simulink model "SimulinkAnalysisofCheetahTail"  (R2022a)
(part 4 of 21)

t1922 = ct{753};
t1923 = ct{754};
t1924 = ct{755};
t1926 = ct{756};
t1928 = ct{757};
t1929 = ct{758};
t1930 = ct{759};
t1931 = ct{760};
t1933 = ct{761};
t1935 = ct{762};
t1937 = ct{763};
t1938 = ct{764};
t1939 = ct{765};
t1940 = ct{766};
t1941 = ct{767};
t1942 = ct{768};
t1943 = ct{769};
t1945 = ct{770};
t1949 = ct{771};
t195 = ct{772};
t1950 = ct{773};
t1951 = ct{774};
t1952 = ct{775};
t1953 = ct{776};
t1955 = ct{777};
t1956 = ct{778};
t1957 = ct{779};
t1959 = ct{780};
t1960 = ct{781};
t1961 = ct{782};
t1962 = ct{783};
t1963 = ct{784};
t1964 = ct{785};
t1965 = ct{786};
t1966 = ct{787};
t1967 = ct{788};
t1968 = ct{789};
t1969 = ct{790};
t197 = ct{791};
t1970 = ct{792};
t1971 = ct{793};
t1973 = ct{794};
t1974 = ct{795};
t1975 = ct{796};
t1976 = ct{797};
t1977 = ct{798};
t1978 = ct{799};
t1979 = ct{800};
t1980 = ct{801};
t1981 = ct{802};
t1982 = ct{803};
t1983 = ct{804};
t1984 = ct{805};
t1985 = ct{806};
t1986 = ct{807};
t1987 = ct{808};
t1988 = ct{809};
t1989 = ct{810};
t1990 = ct{811};
t1992 = ct{812};
t1993 = ct{813};
t1994 = ct{814};
t1995 = ct{815};
t1996 = ct{816};
t1998 = ct{817};
t1999 = ct{818};
t2 = ct{819};
t2000 = ct{820};
t2004 = ct{821};
t2005 = ct{822};
t2006 = ct{823};
t2007 = ct{824};
t2008 = ct{825};
t2009 = ct{826};
t2014 = ct{827};
t2015 = ct{828};
t2016 = ct{829};
t2017 = ct{830};
t2018 = ct{831};
t2020 = ct{832};
t2022 = ct{833};
t2023 = ct{834};
t2024 = ct{835};
t2025 = ct{836};
t2026 = ct{837};
t2027 = ct{838};
t2028 = ct{839};
t2030 = ct{840};
t2033 = ct{841};
t2035 = ct{842};
t2036 = ct{843};
t2037 = ct{844};
t2041 = ct{845};
t2042 = ct{846};
t2043 = ct{847};
t2045 = ct{848};
t2046 = ct{849};
t2047 = ct{850};
t2048 = ct{851};
t2049 = ct{852};
t2050 = ct{853};
t2052 = ct{854};
t2053 = ct{855};
t2056 = ct{856};
t2057 = ct{857};
t2058 = ct{858};
t2059 = ct{859};
t2060 = ct{860};
t2061 = ct{861};
t2062 = ct{862};
t2063 = ct{863};
t2064 = ct{864};
t2065 = ct{865};
t2066 = ct{866};
t2067 = ct{867};
t2068 = ct{868};
t2069 = ct{869};
t2070 = ct{870};
t2072 = ct{871};
t2074 = ct{872};
t2075 = ct{873};
t2076 = ct{874};
t2077 = ct{875};
t2078 = ct{876};
t2079 = ct{877};
t2081 = ct{878};
t2082 = ct{879};
t2083 = ct{880};
t2084 = ct{881};
t2087 = ct{882};
t2088 = ct{883};
t2090 = ct{884};
t2091 = ct{885};
t2092 = ct{886};
t2094 = ct{887};
t2095 = ct{888};
t2096 = ct{889};
t2097 = ct{890};
t2098 = ct{891};
t2099 = ct{892};
t2100 = ct{893};
t2102 = ct{894};
t2103 = ct{895};
t2104 = ct{896};
t2105 = ct{897};
t2106 = ct{898};
t2108 = ct{899};
t2109 = ct{900};
t2110 = ct{901};
t2113 = ct{902};
t2114 = ct{903};
t2116 = ct{904};
t2117 = ct{905};
t2118 = ct{906};
t2119 = ct{907};
t2120 = ct{908};
t2121 = ct{909};
t2123 = ct{910};
t2124 = ct{911};
t2126 = ct{912};
t2127 = ct{913};
t2129 = ct{914};
t2130 = ct{915};
t2131 = ct{916};
t2132 = ct{917};
t2134 = ct{918};
t2135 = ct{919};
t2136 = ct{920};
t2137 = ct{921};
t214 = ct{922};
t2141 = ct{923};
t2142 = ct{924};
t2143 = ct{925};
t2144 = ct{926};
t2146 = ct{927};
t2147 = ct{928};
t2148 = ct{929};
t2149 = ct{930};
t2150 = ct{931};
t2151 = ct{932};
t2152 = ct{933};
t2153 = ct{934};
t2154 = ct{935};
t2155 = ct{936};
t2156 = ct{937};
t2157 = ct{938};
t2158 = ct{939};
t2161 = ct{940};
t2163 = ct{941};
t2165 = ct{942};
t2167 = ct{943};
t2168 = ct{944};
t2171 = ct{945};
t2172 = ct{946};
t2174 = ct{947};
t2176 = ct{948};
t2178 = ct{949};
t2179 = ct{950};
t2181 = ct{951};
t2182 = ct{952};
t2183 = ct{953};
t2184 = ct{954};
t2186 = ct{955};
t2187 = ct{956};
t2188 = ct{957};
t2189 = ct{958};
t2190 = ct{959};
t2191 = ct{960};
t2192 = ct{961};
t2196 = ct{962};
t2199 = ct{963};
t2201 = ct{964};
t2202 = ct{965};
t2203 = ct{966};
t2205 = ct{967};
t2206 = ct{968};
t2208 = ct{969};
t2209 = ct{970};
t2211 = ct{971};
t2212 = ct{972};
t2213 = ct{973};
t2214 = ct{974};
t2215 = ct{975};
t2216 = ct{976};
t2217 = ct{977};
t2218 = ct{978};
t2219 = ct{979};
t2220 = ct{980};
t2221 = ct{981};
t2222 = ct{982};
t2223 = ct{983};
t2224 = ct{984};
t2225 = ct{985};
t2227 = ct{986};
t2228 = ct{987};
t2229 = ct{988};
t2230 = ct{989};
t2231 = ct{990};
t2232 = ct{991};
t2233 = ct{992};
t2235 = ct{993};
t2237 = ct{994};
t2238 = ct{995};
t2239 = ct{996};
t2240 = ct{997};
t2242 = ct{998};
t2245 = ct{999};
t2246 = ct{1000};
t2247 = ct{1001};
t2248 = ct{1002};
t2249 = ct{1003};
t2251 = ct{1004};
t2252 = ct{1005};
t2253 = ct{1006};
t2254 = ct{1007};
t2255 = ct{1008};
t2257 = ct{1009};
t2258 = ct{1010};
t2259 = ct{1011};
t2260 = ct{1012};
t2262 = ct{1013};
t2263 = ct{1014};
t2265 = ct{1015};
t2267 = ct{1016};
t2268 = ct{1017};
t2269 = ct{1018};
t2271 = ct{1019};
t2272 = ct{1020};
t2273 = ct{1021};
t2274 = ct{1022};
t2276 = ct{1023};
t2277 = ct{1024};
t2281 = ct{1025};
t2285 = ct{1026};
t2286 = ct{1027};
t2287 = ct{1028};
t2288 = ct{1029};
t2289 = ct{1030};
t2290 = ct{1031};
t2292 = ct{1032};
t2293 = ct{1033};
t2294 = ct{1034};
t2296 = ct{1035};
t2298 = ct{1036};
t2299 = ct{1037};
t2301 = ct{1038};
t2303 = ct{1039};
t2304 = ct{1040};
t2305 = ct{1041};
t2307 = ct{1042};
t2308 = ct{1043};
t2309 = ct{1044};
t2312 = ct{1045};
t2314 = ct{1046};
t2316 = ct{1047};
t2317 = ct{1048};
t2318 = ct{1049};
t2319 = ct{1050};
t2320 = ct{1051};
t2321 = ct{1052};
t2322 = ct{1053};
t2323 = ct{1054};
t2324 = ct{1055};
t2325 = ct{1056};
t2326 = ct{1057};
t2327 = ct{1058};
t2328 = ct{1059};
t2330 = ct{1060};
t2331 = ct{1061};
t2334 = ct{1062};
t2335 = ct{1063};
t2336 = ct{1064};
t2338 = ct{1065};
t2339 = ct{1066};
t2340 = ct{1067};
t2341 = ct{1068};
t2342 = ct{1069};
t2343 = ct{1070};
t2344 = ct{1071};
t2345 = ct{1072};
t2346 = ct{1073};
t2347 = ct{1074};
t2348 = ct{1075};
t2349 = ct{1076};
t2350 = ct{1077};
t2351 = ct{1078};
t2352 = ct{1079};
t2353 = ct{1080};
t2354 = ct{1081};
t2356 = ct{1082};
t2357 = ct{1083};
t2358 = ct{1084};
t2360 = ct{1085};
t2361 = ct{1086};
t2362 = ct{1087};
t2363 = ct{1088};
t2364 = ct{1089};
t2365 = ct{1090};
t2369 = ct{1091};
t2371 = ct{1092};
t2373 = ct{1093};
t2375 = ct{1094};
t2376 = ct{1095};
t2377 = ct{1096};
t2378 = ct{1097};
t2380 = ct{1098};
t2381 = ct{1099};
t2382 = ct{1100};
t2385 = ct{1101};
t2386 = ct{1102};
t2387 = ct{1103};
t2388 = ct{1104};
t2389 = ct{1105};
t2390 = ct{1106};
t2392 = ct{1107};
t2396 = ct{1108};
t2397 = ct{1109};
t2399 = ct{1110};
t24 = ct{1111};
t2400 = ct{1112};
t2401 = ct{1113};
t2403 = ct{1114};
t2404 = ct{1115};
t2406 = ct{1116};
t2407 = ct{1117};
t2408 = ct{1118};
t2409 = ct{1119};
t2411 = ct{1120};
t2412 = ct{1121};
t2414 = ct{1122};
t2415 = ct{1123};
t2417 = ct{1124};
t2418 = ct{1125};
t2419 = ct{1126};
t2420 = ct{1127};
t2422 = ct{1128};
t2423 = ct{1129};
t2425 = ct{1130};
t2426 = ct{1131};
t2427 = ct{1132};
t2428 = ct{1133};
t2429 = ct{1134};
t2430 = ct{1135};
t2431 = ct{1136};
t2432 = ct{1137};
t2433 = ct{1138};
t2434 = ct{1139};
t2435 = ct{1140};
t2436 = ct{1141};
t2437 = ct{1142};
t2438 = ct{1143};
t2439 = ct{1144};
t2440 = ct{1145};
t2441 = ct{1146};
t2442 = ct{1147};
t2443 = ct{1148};
t2445 = ct{1149};
t2446 = ct{1150};
t2447 = ct{1151};
t2449 = ct{1152};
t2453 = ct{1153};
t2455 = ct{1154};
t2458 = ct{1155};
t2460 = ct{1156};
t2461 = ct{1157};
t2462 = ct{1158};
t2463 = ct{1159};
t2464 = ct{1160};
t2465 = ct{1161};
t2466 = ct{1162};
t2467 = ct{1163};
t2468 = ct{1164};
t2469 = ct{1165};
t2470 = ct{1166};
t2471 = ct{1167};
t2472 = ct{1168};
t2474 = ct{1169};
t2476 = ct{1170};
t2479 = ct{1171};
t2480 = ct{1172};
t2483 = ct{1173};
t2484 = ct{1174};
t2485 = ct{1175};
t2486 = ct{1176};
t2487 = ct{1177};
t2488 = ct{1178};
t2489 = ct{1179};
t2492 = ct{1180};
t2495 = ct{1181};
t2499 = ct{1182};
t25 = ct{1183};
t2502 = ct{1184};
t2503 = ct{1185};
t2504 = ct{1186};
t2505 = ct{1187};
t2506 = ct{1188};
t2507 = ct{1189};
t2509 = ct{1190};
t2511 = ct{1191};
t2512 = ct{1192};
t2513 = ct{1193};
t2514 = ct{1194};
t2515 = ct{1195};
t2516 = ct{1196};
t2518 = ct{1197};
t2519 = ct{1198};
t2520 = ct{1199};
t2521 = ct{1200};
t2522 = ct{1201};
t2523 = ct{1202};
t2524 = ct{1203};
t2525 = ct{1204};
t2526 = ct{1205};
t2527 = ct{1206};
t2528 = ct{1207};
t2529 = ct{1208};
t2530 = ct{1209};
t2531 = ct{1210};
t2532 = ct{1211};
t2533 = ct{1212};
t2534 = ct{1213};
t2535 = ct{1214};
t2536 = ct{1215};
t2539 = ct{1216};
t2540 = ct{1217};
t2541 = ct{1218};
t2542 = ct{1219};
t2543 = ct{1220};
t2544 = ct{1221};
t2545 = ct{1222};
t2546 = ct{1223};
t2547 = ct{1224};
t2550 = ct{1225};
t2551 = ct{1226};
t2552 = ct{1227};
t2560 = ct{1228};
t2561 = ct{1229};
t2562 = ct{1230};
t2563 = ct{1231};
t2564 = ct{1232};
t2565 = ct{1233};
t2566 = ct{1234};
t2567 = ct{1235};
t2568 = ct{1236};
t2569 = ct{1237};
t2570 = ct{1238};
t2571 = ct{1239};
t2576 = ct{1240};
t2577 = ct{1241};
t2579 = ct{1242};
t2580 = ct{1243};
t2581 = ct{1244};
t2582 = ct{1245};
t2584 = ct{1246};
t2587 = ct{1247};
t2588 = ct{1248};
t2589 = ct{1249};
t259 = ct{1250};
t2590 = ct{1251};
t2591 = ct{1252};
t2596 = ct{1253};
t2597 = ct{1254};
t2598 = ct{1255};
t2599 = ct{1256};
t26 = ct{1257};
t260 = ct{1258};
t2600 = ct{1259};
t2605 = ct{1260};
t2607 = ct{1261};
t2610 = ct{1262};
t2611 = ct{1263};
t2612 = ct{1264};
t2613 = ct{1265};
t2614 = ct{1266};
t2615 = ct{1267};
t2616 = ct{1268};
t2617 = ct{1269};
t2618 = ct{1270};
t2619 = ct{1271};
t2620 = ct{1272};
t2621 = ct{1273};
t2622 = ct{1274};
t2623 = ct{1275};
t2624 = ct{1276};
t2627 = ct{1277};
t2629 = ct{1278};
t2631 = ct{1279};
t2632 = ct{1280};
t2634 = ct{1281};
t2635 = ct{1282};
t2636 = ct{1283};
t2637 = ct{1284};
t2638 = ct{1285};
t2640 = ct{1286};
t2641 = ct{1287};
t2643 = ct{1288};
t2646 = ct{1289};
t2647 = ct{1290};
t2648 = ct{1291};
t2649 = ct{1292};
t2650 = ct{1293};
t2654 = ct{1294};
t2656 = ct{1295};
t2657 = ct{1296};
t2658 = ct{1297};
t2660 = ct{1298};
t2662 = ct{1299};
t2663 = ct{1300};
t2664 = ct{1301};
t2665 = ct{1302};
t2666 = ct{1303};
t2667 = ct{1304};
t2668 = ct{1305};
t2669 = ct{1306};
t2671 = ct{1307};
t2673 = ct{1308};
t2677 = ct{1309};
t2678 = ct{1310};
t2679 = ct{1311};
t2681 = ct{1312};
t2682 = ct{1313};
t2683 = ct{1314};
t2684 = ct{1315};
t2688 = ct{1316};
t2689 = ct{1317};
t2691 = ct{1318};
t2692 = ct{1319};
t2695 = ct{1320};
t2696 = ct{1321};
t2698 = ct{1322};
t2699 = ct{1323};
t27 = ct{1324};
t2700 = ct{1325};
t2702 = ct{1326};
t2703 = ct{1327};
t2704 = ct{1328};
t2705 = ct{1329};
t2706 = ct{1330};
t2707 = ct{1331};
t2708 = ct{1332};
t2710 = ct{1333};
t2711 = ct{1334};
t2712 = ct{1335};
t2714 = ct{1336};
t2715 = ct{1337};
t2717 = ct{1338};
t2718 = ct{1339};
t2722 = ct{1340};
t2723 = ct{1341};
t2725 = ct{1342};
t2727 = ct{1343};
t2730 = ct{1344};
t2731 = ct{1345};
t2732 = ct{1346};
t2733 = ct{1347};
t2735 = ct{1348};
t2736 = ct{1349};
t2738 = ct{1350};
t2739 = ct{1351};
t2740 = ct{1352};
t2742 = ct{1353};
t2743 = ct{1354};
t2744 = ct{1355};
t2745 = ct{1356};
t2746 = ct{1357};
t2747 = ct{1358};
t2748 = ct{1359};
t2749 = ct{1360};
t2750 = ct{1361};
t2751 = ct{1362};
t2752 = ct{1363};
t2754 = ct{1364};
t2755 = ct{1365};
t2756 = ct{1366};
t2758 = ct{1367};
t2759 = ct{1368};
t276 = ct{1369};
t2760 = ct{1370};
t2761 = ct{1371};
t2762 = ct{1372};
t2763 = ct{1373};
t2764 = ct{1374};
t2765 = ct{1375};
t2766 = ct{1376};
t2768 = ct{1377};
t2769 = ct{1378};
t277 = ct{1379};
t2770 = ct{1380};
t2771 = ct{1381};
t2772 = ct{1382};
t2774 = ct{1383};
t2775 = ct{1384};
t2776 = ct{1385};
t2778 = ct{1386};
t2781 = ct{1387};
t2782 = ct{1388};
t2783 = ct{1389};
t2784 = ct{1390};
t2785 = ct{1391};
t2786 = ct{1392};
t2787 = ct{1393};
t2788 = ct{1394};
t2790 = ct{1395};
t2791 = ct{1396};
t2792 = ct{1397};
t2793 = ct{1398};
t2795 = ct{1399};
t2797 = ct{1400};
t2799 = ct{1401};
t28 = ct{1402};
t2800 = ct{1403};
t2802 = ct{1404};
t2803 = ct{1405};
t2804 = ct{1406};
t2806 = ct{1407};
t2807 = ct{1408};
t2811 = ct{1409};
t2813 = ct{1410};
t2816 = ct{1411};
t2817 = ct{1412};
t2818 = ct{1413};
t2819 = ct{1414};
t2821 = ct{1415};
t2822 = ct{1416};
t2823 = ct{1417};
t2824 = ct{1418};
t2825 = ct{1419};
t2826 = ct{1420};
t2827 = ct{1421};
t2828 = ct{1422};
t283 = ct{1423};
t2830 = ct{1424};
t2831 = ct{1425};
t2832 = ct{1426};
t2833 = ct{1427};
t2834 = ct{1428};
t2835 = ct{1429};
t2836 = ct{1430};
t2837 = ct{1431};
t2838 = ct{1432};
t2839 = ct{1433};
t284 = ct{1434};
t2841 = ct{1435};
t2842 = ct{1436};
t2843 = ct{1437};
t2844 = ct{1438};
t2845 = ct{1439};
t2846 = ct{1440};
t2847 = ct{1441};
t2849 = ct{1442};
t285 = ct{1443};
t2850 = ct{1444};
t2851 = ct{1445};
t2853 = ct{1446};
t2857 = ct{1447};
t2859 = ct{1448};
t286 = ct{1449};
t2860 = ct{1450};
t2862 = ct{1451};
t2864 = ct{1452};
t2865 = ct{1453};
t2866 = ct{1454};
t2867 = ct{1455};
t2869 = ct{1456};
t287 = ct{1457};
t2870 = ct{1458};
t2871 = ct{1459};
t2872 = ct{1460};
t2874 = ct{1461};
t2875 = ct{1462};
t2876 = ct{1463};
t2877 = ct{1464};
t2878 = ct{1465};
t2879 = ct{1466};
t288 = ct{1467};
t2880 = ct{1468};
t2881 = ct{1469};
t2882 = ct{1470};
t2883 = ct{1471};
t2884 = ct{1472};
t2885 = ct{1473};
t2886 = ct{1474};
t2887 = ct{1475};
t2889 = ct{1476};
t289 = ct{1477};
t2890 = ct{1478};
t2892 = ct{1479};
t2895 = ct{1480};
t2896 = ct{1481};
t2897 = ct{1482};
t2898 = ct{1483};
t2899 = ct{1484};
t290 = ct{1485};
t2900 = ct{1486};
t2902 = ct{1487};
t2903 = ct{1488};
t2906 = ct{1489};
t2907 = ct{1490};
t2909 = ct{1491};
t291 = ct{1492};
t2912 = ct{1493};
t2913 = ct{1494};
t2914 = ct{1495};
t2915 = ct{1496};
t2916 = ct{1497};
t2917 = ct{1498};
t2918 = ct{1499};
t2919 = ct{1500};
t292 = ct{1501};
t2920 = ct{1502};
t2923 = ct{1503};
t2924 = ct{1504};
t2926 = ct{1505};
t2927 = ct{1506};
t2928 = ct{1507};
t2929 = ct{1508};
t293 = ct{1509};
t2931 = ct{1510};
t2932 = ct{1511};
t2935 = ct{1512};
t2938 = ct{1513};
t294 = ct{1514};
t2940 = ct{1515};
t2942 = ct{1516};
t2943 = ct{1517};
t2944 = ct{1518};
t2945 = ct{1519};
t2946 = ct{1520};
t2947 = ct{1521};
t2949 = ct{1522};
t2950 = ct{1523};
t2951 = ct{1524};
t2952 = ct{1525};
t2953 = ct{1526};
t2954 = ct{1527};
t2955 = ct{1528};
t2956 = ct{1529};
t2957 = ct{1530};
t2959 = ct{1531};
t2960 = ct{1532};
t2961 = ct{1533};
t2962 = ct{1534};
t2963 = ct{1535};
t2964 = ct{1536};
t2966 = ct{1537};
t2967 = ct{1538};
t2969 = ct{1539};
t2972 = ct{1540};
t2975 = ct{1541};
t2976 = ct{1542};
t2977 = ct{1543};
t2978 = ct{1544};
t2979 = ct{1545};
t2981 = ct{1546};
t2982 = ct{1547};
t2985 = ct{1548};
t2988 = ct{1549};
t2989 = ct{1550};
t2992 = ct{1551};
t2994 = ct{1552};
t2995 = ct{1553};
t2996 = ct{1554};
t2998 = ct{1555};
t3 = ct{1556};
t30 = ct{1557};
t3003 = ct{1558};
t3004 = ct{1559};
t3006 = ct{1560};
t3007 = ct{1561};
t3008 = ct{1562};
t3009 = ct{1563};
t3010 = ct{1564};
t3011 = ct{1565};
t3012 = ct{1566};
t3014 = ct{1567};
t3015 = ct{1568};
t3016 = ct{1569};
t3017 = ct{1570};
t3019 = ct{1571};
t3020 = ct{1572};
t3021 = ct{1573};
t3022 = ct{1574};
t3023 = ct{1575};
t3025 = ct{1576};
t3026 = ct{1577};
t3027 = ct{1578};
t3028 = ct{1579};
t3030 = ct{1580};
t3031 = ct{1581};
t3033 = ct{1582};
t3034 = ct{1583};
t3035 = ct{1584};
t3036 = ct{1585};
t3037 = ct{1586};
t3038 = ct{1587};
t3039 = ct{1588};
t304 = ct{1589};
t3041 = ct{1590};
t3042 = ct{1591};
t3043 = ct{1592};
t3044 = ct{1593};
t3045 = ct{1594};
t3046 = ct{1595};
t3047 = ct{1596};
t3048 = ct{1597};
t3050 = ct{1598};
t3051 = ct{1599};
t3054 = ct{1600};
t3057 = ct{1601};
t3059 = ct{1602};
t3060 = ct{1603};
t3061 = ct{1604};
t3062 = ct{1605};
t3063 = ct{1606};
t3064 = ct{1607};
t3065 = ct{1608};
t3066 = ct{1609};
t3069 = ct{1610};
t3070 = ct{1611};
t3072 = ct{1612};
t3074 = ct{1613};
t3075 = ct{1614};
t3077 = ct{1615};
t3078 = ct{1616};
t3081 = ct{1617};
t3082 = ct{1618};
t3083 = ct{1619};
t3084 = ct{1620};
t3085 = ct{1621};
t3087 = ct{1622};
t3089 = ct{1623};
t3090 = ct{1624};
t3091 = ct{1625};
t3092 = ct{1626};
t3093 = ct{1627};
t3094 = ct{1628};
t3095 = ct{1629};
t3097 = ct{1630};
t3098 = ct{1631};
t3099 = ct{1632};
t3100 = ct{1633};
t3102 = ct{1634};
t3105 = ct{1635};
t3106 = ct{1636};
t3107 = ct{1637};
t3108 = ct{1638};
t3109 = ct{1639};
t3110 = ct{1640};
t3112 = ct{1641};
t3113 = ct{1642};
t3114 = ct{1643};
t3115 = ct{1644};
t3117 = ct{1645};
t3119 = ct{1646};
t3122 = ct{1647};
t3124 = ct{1648};
t3127 = ct{1649};
t3128 = ct{1650};
t3129 = ct{1651};
t3130 = ct{1652};
t3131 = ct{1653};
t3132 = ct{1654};
t3133 = ct{1655};
t3134 = ct{1656};
t3135 = ct{1657};
t3136 = ct{1658};
t3138 = ct{1659};
t3142 = ct{1660};
t3143 = ct{1661};
t3145 = ct{1662};
t3146 = ct{1663};
t3147 = ct{1664};
t3149 = ct{1665};
t3151 = ct{1666};
t3153 = ct{1667};
t3154 = ct{1668};
t3157 = ct{1669};
t3158 = ct{1670};
t3160 = ct{1671};
t3162 = ct{1672};
t3164 = ct{1673};
t3165 = ct{1674};
t3166 = ct{1675};
t3167 = ct{1676};
t3169 = ct{1677};
t3170 = ct{1678};
t3171 = ct{1679};
t3173 = ct{1680};
t3174 = ct{1681};
t3175 = ct{1682};
t3176 = ct{1683};
t3177 = ct{1684};
t3179 = ct{1685};
t3180 = ct{1686};
t3181 = ct{1687};
t3184 = ct{1688};
t3186 = ct{1689};
t3187 = ct{1690};
t3189 = ct{1691};
t3195 = ct{1692};
t3197 = ct{1693};
t3199 = ct{1694};
t3200 = ct{1695};
t3203 = ct{1696};
t3204 = ct{1697};
t3207 = ct{1698};
t3210 = ct{1699};
t3212 = ct{1700};
t3213 = ct{1701};
t3216 = ct{1702};
t3217 = ct{1703};
t3218 = ct{1704};
t3220 = ct{1705};
t3221 = ct{1706};
t3222 = ct{1707};
t3223 = ct{1708};
t3224 = ct{1709};
t3226 = ct{1710};
t3228 = ct{1711};
t3229 = ct{1712};
t3230 = ct{1713};
t3233 = ct{1714};
t3235 = ct{1715};
t3236 = ct{1716};
t3237 = ct{1717};
t3238 = ct{1718};
t3239 = ct{1719};
t3240 = ct{1720};
t3241 = ct{1721};
t3243 = ct{1722};
t3244 = ct{1723};
t3245 = ct{1724};
t3246 = ct{1725};
t3247 = ct{1726};
t3248 = ct{1727};
t3249 = ct{1728};
t3252 = ct{1729};
t3256 = ct{1730};
t3260 = ct{1731};
t3263 = ct{1732};
t3265 = ct{1733};
t3266 = ct{1734};
t3270 = ct{1735};
t3272 = ct{1736};
t3273 = ct{1737};
t3274 = ct{1738};
t3275 = ct{1739};
t3277 = ct{1740};
t3278 = ct{1741};
t3279 = ct{1742};
t3280 = ct{1743};
t3281 = ct{1744};
t3282 = ct{1745};
t3284 = ct{1746};
t3285 = ct{1747};
t3286 = ct{1748};
t3287 = ct{1749};
t3290 = ct{1750};
t3291 = ct{1751};
t3294 = ct{1752};
t3295 = ct{1753};
t3296 = ct{1754};
t3298 = ct{1755};
t33 = ct{1756};
t3301 = ct{1757};
t3303 = ct{1758};
t3304 = ct{1759};
t3305 = ct{1760};
t3306 = ct{1761};
t3307 = ct{1762};
t3309 = ct{1763};
t3315 = ct{1764};
t3317 = ct{1765};
t3319 = ct{1766};
t3321 = ct{1767};
t3322 = ct{1768};
t3323 = ct{1769};
t3325 = ct{1770};
t3330 = ct{1771};
t3331 = ct{1772};
t3332 = ct{1773};
t3333 = ct{1774};
t3337 = ct{1775};
t3339 = ct{1776};
t3341 = ct{1777};
t3345 = ct{1778};
t3351 = ct{1779};
t3353 = ct{1780};
t3357 = ct{1781};
t3359 = ct{1782};
t3360 = ct{1783};
t3361 = ct{1784};
t3362 = ct{1785};
t3364 = ct{1786};
t3366 = ct{1787};
t3368 = ct{1788};
t3369 = ct{1789};
t3370 = ct{1790};
t3372 = ct{1791};
t3373 = ct{1792};
t3376 = ct{1793};
t3378 = ct{1794};
t3379 = ct{1795};
t3380 = ct{1796};
t3381 = ct{1797};
t3384 = ct{1798};
t3385 = ct{1799};
t3389 = ct{1800};
t3390 = ct{1801};
t3391 = ct{1802};
t3392 = ct{1803};
t3393 = ct{1804};
t3395 = ct{1805};
t3397 = ct{1806};
t3399 = ct{1807};
t34 = ct{1808};
t3403 = ct{1809};
t3412 = ct{1810};
t3415 = ct{1811};
t3416 = ct{1812};
t3418 = ct{1813};
t3419 = ct{1814};
t3420 = ct{1815};
t3422 = ct{1816};
t3425 = ct{1817};
t3426 = ct{1818};
t3427 = ct{1819};
t3429 = ct{1820};
t3434 = ct{1821};
t3436 = ct{1822};
t3437 = ct{1823};
t3438 = ct{1824};
t3441 = ct{1825};
t3446 = ct{1826};
t3447 = ct{1827};
t3448 = ct{1828};
t3449 = ct{1829};
t3450 = ct{1830};
t3451 = ct{1831};
t3453 = ct{1832};
t3454 = ct{1833};
t3457 = ct{1834};
t3459 = ct{1835};
t3460 = ct{1836};
t3461 = ct{1837};
t3468 = ct{1838};
t3469 = ct{1839};
t3471 = ct{1840};
t3474 = ct{1841};
t3478 = ct{1842};
t3483 = ct{1843};
t3484 = ct{1844};
t3487 = ct{1845};
t3488 = ct{1846};
t3490 = ct{1847};
t3492 = ct{1848};
t3493 = ct{1849};
t3495 = ct{1850};
t3498 = ct{1851};
t3499 = ct{1852};
t35 = ct{1853};
t3500 = ct{1854};
t3501 = ct{1855};
t3502 = ct{1856};
t3504 = ct{1857};
t3507 = ct{1858};
t3512 = ct{1859};
t3514 = ct{1860};
t3516 = ct{1861};
t3520 = ct{1862};
t3521 = ct{1863};
t3522 = ct{1864};
t3523 = ct{1865};
t3524 = ct{1866};
t3525 = ct{1867};
t3527 = ct{1868};
t3528 = ct{1869};
t3529 = ct{1870};
t3530 = ct{1871};
t3531 = ct{1872};
t3536 = ct{1873};
t3539 = ct{1874};
t3542 = ct{1875};
t3543 = ct{1876};
t3545 = ct{1877};
t3546 = ct{1878};
t3547 = ct{1879};
t3548 = ct{1880};
t3549 = ct{1881};
t3551 = ct{1882};
t3559 = ct{1883};
t3560 = ct{1884};
t3561 = ct{1885};
t3562 = ct{1886};
t3564 = ct{1887};
t3565 = ct{1888};
t3566 = ct{1889};
t3567 = ct{1890};
t3568 = ct{1891};
t3569 = ct{1892};
t3570 = ct{1893};
t3571 = ct{1894};
t3572 = ct{1895};
t3573 = ct{1896};
t3574 = ct{1897};
t3576 = ct{1898};
t3579 = ct{1899};
t3581 = ct{1900};
t3583 = ct{1901};
t3584 = ct{1902};
t3590 = ct{1903};
t3595 = ct{1904};
t3596 = ct{1905};
t3598 = ct{1906};
t3609 = ct{1907};
t3611 = ct{1908};
t3612 = ct{1909};
t3614 = ct{1910};
t3617 = ct{1911};
t3619 = ct{1912};
t3621 = ct{1913};
t3626 = ct{1914};
t3627 = ct{1915};
t3628 = ct{1916};
t3630 = ct{1917};
t3632 = ct{1918};
t3635 = ct{1919};
t3636 = ct{1920};
t3637 = ct{1921};
t3638 = ct{1922};
t3639 = ct{1923};
t3641 = ct{1924};
t3642 = ct{1925};
t3643 = ct{1926};
t3644 = ct{1927};
t3647 = ct{1928};
t3649 = ct{1929};
t3651 = ct{1930};
t3652 = ct{1931};
t3655 = ct{1932};
t3656 = ct{1933};
t3657 = ct{1934};
t3659 = ct{1935};
t3662 = ct{1936};
t3663 = ct{1937};
t3666 = ct{1938};
t3671 = ct{1939};
t3672 = ct{1940};
t3677 = ct{1941};
t3678 = ct{1942};
t3679 = ct{1943};
t3680 = ct{1944};
t3683 = ct{1945};
t3684 = ct{1946};
t3686 = ct{1947};
t3687 = ct{1948};
t3696 = ct{1949};
t3698 = ct{1950};
t3699 = ct{1951};
t3700 = ct{1952};
t3701 = ct{1953};
t3702 = ct{1954};
t3703 = ct{1955};
t3704 = ct{1956};
t3706 = ct{1957};
t3708 = ct{1958};
t3709 = ct{1959};
t3710 = ct{1960};
t3713 = ct{1961};
t3716 = ct{1962};
t3717 = ct{1963};
t3721 = ct{1964};
t3722 = ct{1965};
t3724 = ct{1966};
t3726 = ct{1967};
t3730 = ct{1968};
t3739 = ct{1969};
t3743 = ct{1970};
t3749 = ct{1971};
t375 = ct{1972};
t3750 = ct{1973};
t3752 = ct{1974};
t376 = ct{1975};
t3761 = ct{1976};
t3768 = ct{1977};
t3769 = ct{1978};
t377 = ct{1979};
t3771 = ct{1980};
t3772 = ct{1981};
t3787 = ct{1982};
t3790 = ct{1983};
t3791 = ct{1984};
t3792 = ct{1985};
t38 = ct{1986};
t381 = ct{1987};
t3819 = ct{1988};
t382 = ct{1989};
t3823 = ct{1990};
t3828 = ct{1991};
t383 = ct{1992};
t3832 = ct{1993};
t3835 = ct{1994};
t3842 = ct{1995};
t3847 = ct{1996};
t3855 = ct{1997};
t3858 = ct{1998};
t3862 = ct{1999};
t3866 = ct{2000};
t3873 = ct{2001};
t3880 = ct{2002};
t3882 = ct{2003};
t3883 = ct{2004};
t390 = ct{2005};
t3900 = ct{2006};
t3902 = ct{2007};
t3906 = ct{2008};
t3907 = ct{2009};
t3908 = ct{2010};
t3909 = ct{2011};
t3910 = ct{2012};
t3913 = ct{2013};
t3915 = ct{2014};
t3916 = ct{2015};
t3926 = ct{2016};
t3928 = ct{2017};
t3929 = ct{2018};
t3930 = ct{2019};
t3931 = ct{2020};
t3932 = ct{2021};
t3933 = ct{2022};
t3936 = ct{2023};
t3937 = ct{2024};
t394 = ct{2025};
t3940 = ct{2026};
t3942 = ct{2027};
t3944 = ct{2028};
t3952 = ct{2029};
t3955 = ct{2030};
t3956 = ct{2031};
t3957 = ct{2032};
t3959 = ct{2033};
t3960 = ct{2034};
t3961 = ct{2035};
t3962 = ct{2036};
t3964 = ct{2037};
t3965 = ct{2038};
t3967 = ct{2039};
t3968 = ct{2040};
t3969 = ct{2041};
t3971 = ct{2042};
t3974 = ct{2043};
t3976 = ct{2044};
t3981 = ct{2045};
t3982 = ct{2046};
t3983 = ct{2047};
t3993 = ct{2048};
t3994 = ct{2049};
t3995 = ct{2050};
t3996 = ct{2051};
t3998 = ct{2052};
t4 = ct{2053};
t400 = ct{2054};
t4003 = ct{2055};
t4004 = ct{2056};
t4008 = ct{2057};
t401 = ct{2058};
t4012 = ct{2059};
t4014 = ct{2060};
t4028 = ct{2061};
t4029 = ct{2062};
t4033 = ct{2063};
t4035 = ct{2064};
t4036 = ct{2065};
t4038 = ct{2066};
t4042 = ct{2067};
t4047 = ct{2068};
t4048 = ct{2069};
t4049 = ct{2070};
t4051 = ct{2071};
t4052 = ct{2072};
t4054 = ct{2073};
t4056 = ct{2074};
t4058 = ct{2075};
t4059 = ct{2076};
t4060 = ct{2077};
t4061 = ct{2078};
t4064 = ct{2079};
t4068 = ct{2080};
t4070 = ct{2081};
t4073 = ct{2082};
t4074 = ct{2083};
t4078 = ct{2084};
t4081 = ct{2085};
t4086 = ct{2086};
t4087 = ct{2087};
t4088 = ct{2088};
t4089 = ct{2089};
t4090 = ct{2090};
t4092 = ct{2091};
t4093 = ct{2092};
t4094 = ct{2093};
t4095 = ct{2094};
t4098 = ct{2095};
t4099 = ct{2096};
t41 = ct{2097};
t410 = ct{2098};
t4101 = ct{2099};
t4103 = ct{2100};
t4104 = ct{2101};
t4106 = ct{2102};
t4109 = ct{2103};
t411 = ct{2104};
t4110 = ct{2105};
t4112 = ct{2106};
t4113 = ct{2107};
t4114 = ct{2108};
t4118 = ct{2109};
t4119 = ct{2110};
t412 = ct{2111};
t4121 = ct{2112};
t4124 = ct{2113};
t413 = ct{2114};
t4136 = ct{2115};
t414 = ct{2116};
t4141 = ct{2117};
t4143 = ct{2118};
t4149 = ct{2119};
t415 = ct{2120};
t4153 = ct{2121};
t4155 = ct{2122};
t4156 = ct{2123};
t4159 = ct{2124};
t4164 = ct{2125};
t4169 = ct{2126};
t4171 = ct{2127};
t4182 = ct{2128};
t4185 = ct{2129};
t4188 = ct{2130};
t4189 = ct{2131};
t4190 = ct{2132};
t4196 = ct{2133};
t4197 = ct{2134};
t420 = ct{2135};
t4207 = ct{2136};
t421 = ct{2137};
t4210 = ct{2138};
t4218 = ct{2139};
t4222 = ct{2140};
t4224 = ct{2141};
t4231 = ct{2142};
t4232 = ct{2143};
t4234 = ct{2144};
t4236 = ct{2145};
t425 = ct{2146};
t4253 = ct{2147};
t4256 = ct{2148};
t4269 = ct{2149};
t4282 = ct{2150};
t4290 = ct{2151};
t4295 = ct{2152};
t4298 = ct{2153};
t430 = ct{2154};
t4301 = ct{2155};
t4304 = ct{2156};
t4306 = ct{2157};
t431 = ct{2158};
t4316 = ct{2159};
t4323 = ct{2160};
t433 = ct{2161};
t4330 = ct{2162};
t4332 = ct{2163};
t4335 = ct{2164};
t4342 = ct{2165};
t4349 = ct{2166};
t4354 = ct{2167};
t4355 = ct{2168};
t4356 = ct{2169};
t4358 = ct{2170};
t436 = ct{2171};
t4367 = ct{2172};
t4368 = ct{2173};
t44 = ct{2174};
t4418 = ct{2175};
t4420 = ct{2176};
t4421 = ct{2177};
t4432 = ct{2178};
t445 = ct{2179};
t4454 = ct{2180};
t4457 = ct{2181};
t4458 = ct{2182};
t4475 = ct{2183};
t4479 = ct{2184};
t4481 = ct{2185};
t4492 = ct{2186};
t450 = ct{2187};
t451 = ct{2188};
t4512 = ct{2189};
t456 = ct{2190};
t4581 = ct{2191};
t459 = ct{2192};
t4597 = ct{2193};
t4598 = ct{2194};
t46 = ct{2195};
t4603 = ct{2196};
t465 = ct{2197};
t466 = ct{2198};
t4716 = ct{2199};
t4752 = ct{2200};
t4796 = ct{2201};
t48 = ct{2202};
t482 = ct{2203};
t483 = ct{2204};
t484 = ct{2205};
t485 = ct{2206};
t487 = ct{2207};
t488 = ct{2208};
t49 = ct{2209};
t491 = ct{2210};
t496 = ct{2211};
t4995 = ct{2212};
t5 = ct{2213};
t50 = ct{2214};
t501 = ct{2215};
t502 = ct{2216};
t504 = ct{2217};
t505 = ct{2218};
t51 = ct{2219};
t514 = ct{2220};
t519 = ct{2221};
t523 = ct{2222};
t524 = ct{2223};
t527 = ct{2224};
t530 = ct{2225};
t534 = ct{2226};
t537 = ct{2227};
t539 = ct{2228};
t54 = ct{2229};
t541 = ct{2230};
t542 = ct{2231};
t544 = ct{2232};
t546 = ct{2233};
t547 = ct{2234};
t55 = ct{2235};
t550 = ct{2236};
t553 = ct{2237};
t557 = ct{2238};
t558 = ct{2239};
t559 = ct{2240};
t56 = ct{2241};
t560 = ct{2242};
t57 = ct{2243};
t572 = ct{2244};
t573 = ct{2245};
t574 = ct{2246};
t575 = ct{2247};
t587 = ct{2248};
t59 = ct{2249};
t595 = ct{2250};
t6 = ct{2251};
t603 = ct{2252};
t61 = ct{2253};
t614 = ct{2254};
t623 = ct{2255};
t624 = ct{2256};
t627 = ct{2257};
t628 = ct{2258};
t629 = ct{2259};
t632 = ct{2260};
t634 = ct{2261};
t641 = ct{2262};
t643 = ct{2263};
t644 = ct{2264};
t648 = ct{2265};
t65 = ct{2266};
t650 = ct{2267};
t651 = ct{2268};
t655 = ct{2269};
t657 = ct{2270};
t662 = ct{2271};
t664 = ct{2272};
t665 = ct{2273};
t666 = ct{2274};
t667 = ct{2275};
t668 = ct{2276};
t669 = ct{2277};
t672 = ct{2278};
t674 = ct{2279};
t675 = ct{2280};
t68 = ct{2281};
t69 = ct{2282};
t693 = ct{2283};
t699 = ct{2284};
t7 = ct{2285};
t71 = ct{2286};
t720 = ct{2287};
t721 = ct{2288};
t724 = ct{2289};
t73 = ct{2290};
t731 = ct{2291};
t732 = ct{2292};
t735 = ct{2293};
t736 = ct{2294};
t741 = ct{2295};
t744 = ct{2296};
t746 = ct{2297};
t749 = ct{2298};
t751 = ct{2299};
t752 = ct{2300};
t753 = ct{2301};
t754 = ct{2302};
t755 = ct{2303};
t756 = ct{2304};
t757 = ct{2305};
t759 = ct{2306};
t760 = ct{2307};
t761 = ct{2308};
t762 = ct{2309};
t764 = ct{2310};
t765 = ct{2311};
t769 = ct{2312};
t772 = ct{2313};
t774 = ct{2314};
t776 = ct{2315};
t778 = ct{2316};
t779 = ct{2317};
t792 = ct{2318};
t795 = ct{2319};
t797 = ct{2320};
t799 = ct{2321};
t8 = ct{2322};
t801 = ct{2323};
t802 = ct{2324};
t803 = ct{2325};
t805 = ct{2326};
t806 = ct{2327};
t811 = ct{2328};
t817 = ct{2329};
t818 = ct{2330};
t820 = ct{2331};
t821 = ct{2332};
t823 = ct{2333};
t824 = ct{2334};
t828 = ct{2335};
t830 = ct{2336};
t831 = ct{2337};
t834 = ct{2338};
t837 = ct{2339};
t838 = ct{2340};
t839 = ct{2341};
t841 = ct{2342};
t842 = ct{2343};
t843 = ct{2344};
t844 = ct{2345};
t845 = ct{2346};
t846 = ct{2347};
t847 = ct{2348};
t848 = ct{2349};
t850 = ct{2350};
t851 = ct{2351};
t852 = ct{2352};
t853 = ct{2353};
t854 = ct{2354};
t855 = ct{2355};
t859 = ct{2356};
t862 = ct{2357};
t863 = ct{2358};
t864 = ct{2359};
t865 = ct{2360};
t867 = ct{2361};
t868 = ct{2362};
t870 = ct{2363};
t871 = ct{2364};
t872 = ct{2365};
t874 = ct{2366};
t875 = ct{2367};
t876 = ct{2368};
t877 = ct{2369};
t879 = ct{2370};
t885 = ct{2371};
t886 = ct{2372};
t887 = ct{2373};
t888 = ct{2374};
t889 = ct{2375};
t890 = ct{2376};
t891 = ct{2377};
t892 = ct{2378};
t893 = ct{2379};
t896 = ct{2380};
t897 = ct{2381};
t898 = ct{2382};
t9 = ct{2383};
t900 = ct{2384};
t901 = ct{2385};
t902 = ct{2386};
t903 = ct{2387};
t904 = ct{2388};
t906 = ct{2389};
t907 = ct{2390};
t908 = ct{2391};
t909 = ct{2392};
t912 = ct{2393};
t914 = ct{2394};
t915 = ct{2395};
t916 = ct{2396};
t917 = ct{2397};
t918 = ct{2398};
t919 = ct{2399};
t923 = ct{2400};
t924 = ct{2401};
t925 = ct{2402};
t926 = ct{2403};
t927 = ct{2404};
t928 = ct{2405};
t934 = ct{2406};
t947 = ct{2407};
t948 = ct{2408};
t949 = ct{2409};
t950 = ct{2410};
t951 = ct{2411};
t952 = ct{2412};
t953 = ct{2413};
t954 = ct{2414};
t955 = ct{2415};
t957 = ct{2416};
t964 = ct{2417};
t965 = ct{2418};
t966 = ct{2419};
t970 = ct{2420};
t972 = ct{2421};
t977 = ct{2422};
t979 = ct{2423};
t980 = ct{2424};
t983 = ct{2425};
t985 = ct{2426};
t987 = ct{2427};
t990 = ct{2428};
t991 = ct{2429};
t992 = ct{2430};
t993 = ct{2431};
t994 = ct{2432};
t995 = ct{2433};
t996 = ct{2434};
t3744 = -t3672;
t3746 = t1505.*(t103-t544).*3.367829185e-3;
t3759 = -t3683;
t3775 = t2529.*9.52624335e-4;
t3777 = t2536.*9.52624335e-4;
t3779 = t2529.*3.372816795e-3;
t3780 = t456+t830+t862+t1573;
t3781 = t1505.*(t103-t544).*(-8.56645e-6);
t3782 = t2540.*1.90524867e-3;
t3783 = t1505.*(t214-t541).*(-9.52624335e-4);
t3784 = t2536.*3.372816795e-3;
t3788 = t2540.*6.74563359e-3;
t3789 = t1505.*(t214-t541).*(-3.372816795e-3);
t3793 = -t3743;
t3794 = t2770.*3.36554e-3;
t3795 = t2771.*3.36554e-3;
t3804 = -t3771;
t3805 = -t3772;
t3807 = t2635.*9.52624335e-4;
t3808 = t2635.*3.372816795e-3;
t3814 = t2823.*3.36554e-3;
t3815 = t2824.*3.36554e-3;
t3822 = t2833.*3.36554e-3;
t3830 = t1505.*(t534-t546).*(-6.73108e-3);
t3836 = t46+t123+t484+t627+t735+t1487;
t3838 = t1505.*(t534-t546).*6.73108e-3;
t3839 = t1505.*(t534-t546).*(-3.36554e-3);
t3843 = t2770.*9.52624335e-4;
t3844 = t2771.*9.52624335e-4;
t3845 = t2770.*3.372816795e-3;
t3846 = t2771.*3.372816795e-3;
t3851 = -t3828;
t3854 = t1505.*(t534-t546).*3.36554e-3;
t3859 = -t3835;
t3871 = t2833.*9.52624335e-4;
t3877 = t2833.*3.372816795e-3;
t3889 = -Mt.*t1528.*(t433-t828+T_cg_H.*(t197-t537));
t3898 = t1505.*(t534-t546).*(-9.52624335e-4);
t3899 = t1505.*(t534-t546).*(-1.90524867e-3);
t3904 = t1505.*(t534-t546).*(-3.372816795e-3);
t3905 = t1505.*(t534-t546).*(-6.74563359e-3);
t3918 = t1505.*(t534-t546).*6.74563359e-3;
t3919 = t1505.*(t534-t546).*3.372816795e-3;
t3924 = t3129.*6.73108e-3;
t3939 = t3900./2.0;
t3950 = Mb.*t1487.*t2563;
t3985 = -t3956;
t3999 = t3129.*1.90524867e-3;
t4000 = -t3968;
t4002 = t3129.*6.74563359e-3;
t4005 = -t3974;
t4023 = -t4004;
t4024 = -t3993;
t4045 = -t4028;
t4046 = -t4029;
t4053 = -t4035;
t4055 = -t4036;
t4067 = -t4051;
t4069 = -t4056;
t4071 = t643+t1795+t1805;
t4072 = t648+t1797+t1808;
t4075 = t3523.*3.36554e-3;
t4076 = t3524.*3.36554e-3;
t4079 = t662+t732+t966+t1029+t1102;
t4082 = t550+t801+t1023+t1036+t1043;
t4097 = -t4088;
t4100 = t400+t859+t863+t1170+t1289;
t4122 = -t4103;
t4123 = -t1505.*(-t488+t603+dpsi1.*(t105-t465)+dth2.*(t103-t544));
t4125 = -t4106;
t4126 = dphi1.*t4112;
t4130 = -t4110;
t4134 = t3771.*3.36554e-3;
t4135 = t3772.*3.36554e-3;
t4137 = t3791.*3.36554e-3;
t4140 = -t4119;
t4146 = -t4124;
t4157 = Mt.*t4.*t10.*t4112;
t4158 = Mt.*t5.*t9.*t4112;
t4165 = -t4149;
t4174 = Mt.*t5.*t30.*t4112;
t4175 = Mt.*t5.*t34.*t4112;
t4180 = t1262+t1709+t1767;
t4198 = Mt.*t1531.*t3483;
t4203 = -t4185;
t4211 = t3900.*3.36554e-3;
t4212 = t3906.*3.36554e-3;
t4213 = t3907.*3.36554e-3;
t4217 = t3936.*(-3.36554e-3);
t4225 = Mt.*t381.*t4112;
t4226 = Mt.*t382.*t4112;
t4227 = t1264+t1794+t1837;
t4237 = t990+t1924+t1956;
t4240 = t3900.*9.52624335e-4;
t4241 = t3900.*3.372816795e-3;
t4246 = Mt.*t420.*t4112;
t4247 = Mt.*t421.*t4112;
t4270 = t672+t805+t1227+t1228+t1342;
t4274 = t59+t410+t504+t1126+t1335+t1536;
t4276 = t69+t505+t572+t1130+t1266+t1462;
t4286 = t1085+t2033+t2075;
t4300 = t903.*t4113;
t4312 = -t4301;
t4324 = Mt.*t1528.*t3937;
t4325 = Mt.*t2203.*t3483;
t4326 = t1505.*(-t488+t603+dpsi1.*(t105-t465)+dth2.*(t103-t544)).*(-3.36554e-3);
t4339 = -t4335;
t4348 = Mt.*t3483.*(-t44+t390+t430-t524+t587);
t4364 = -t1505.*(-t550+t693+t972-t1023+dpsi1.*(t214-t541));
t4371 = Mt.*t1381.*t4112;
t4393 = t1505.*t4114;
t4395 = t1430.*t4136;
t4406 = Mt.*t2174.*t3937;
t4424 = Mt.*t1727.*t4112;
t4446 = -Mt.*t3940.*(t431+t909+T_cg_H.*(t195-t634));
t4453 = Mt.*t3940.*(t431+t909+T_cg_H.*(t195-t634));
t4464 = Mt.*t2915.*t3940;
t4477 = -Mt.*t4112.*(t433-t828+T_cg_H.*(t197-t537));
t4487 = t1505.*(-t550+t693+t972-t1023+dpsi1.*(t214-t541)).*(-3.36554e-3);
t4490 = t821+t1475+t1541+t1557+t1613;
t4491 = t1018+t1434+t1446+t1504+t1511;
t4495 = Mt.*t4112.*(t433-t828+T_cg_H.*(t197-t537));
t4496 = -t4479;
t4497 = -t4481;
t4506 = -Mt.*t4112.*(t431+t909+T_cg_H.*(t195-t634));
t4525 = Mt.*t2763.*t4112;
t4538 = Mt.*t2915.*t4112;
t4545 = Mt.*t4112.*(-t120+t425+t519-t651+t765);
t4549 = t1673+t3021+t3028;
t4551 = t1670+t3015+t3025;
t4595 = t1058+t1648+t1651+t1768+t1773;
t4602 = t2326+t3014+t3048;
t4628 = t900+t917+t919+t1776+t1897+t1903;
t4646 = t1081+t1145+t1472+t1533+t1588+t1603;
t4649 = t2056+t3286+t3290;
t4659 = Mt.*t3937.*t4112;
t4665 = Mt.*t3971.*t4112;
t4695 = t1080+t1385+t1429+t1503+t1647+t1832;
t4703 = t1325+t1328+t1427+t1441+t1712+t1772;
t4711 = -ITail.*t3967.*(-t1355+t1789+(t9.*t868.*(t105-t465))./2.0);
t4730 = -ITail.*t3967.*(-t1017+(t1240.*(t105-t465))./2.0+(t903.*(t534-t546))./2.0);
t4732 = ITail.*t3967.*(-t1017+(t1240.*(t105-t465))./2.0+(t903.*(t534-t546))./2.0);
t4739 = t887+t1165+t1270+t1760+t2231+t2353;
t4740 = t890+t1161+t1284+t1770+t2224+t2357;
t4779 = -ITail.*t4164.*(-t1017+(t1240.*(t105-t465))./2.0+(t903.*(t534-t546))./2.0);
t4789 = ITail.*t4164.*(-t1017+(t1240.*(t105-t465))./2.0+(t903.*(t534-t546))./2.0);
t4873 = t948+t1209+t1235+t2273+t2931+t2953;
t4909 = -ITail.*t4454.*(-t1355+t1789+(t9.*t868.*(t105-t465))./2.0);
t4925 = -ITail.*t4454.*(-t1017+(t1240.*(t105-t465))./2.0+(t903.*(t534-t546))./2.0);
t4931 = ITail.*(-t1355+t1789+(t9.*t868.*(t105-t465))./2.0).*(-t1018+t1426+t1431-t1446+t3.*t496.*(t105-t465));
t4932 = ITail.*(-t1262+t1701+t9.*t868.*(t105-t465)).*(-t993+t1535+t1540-t1552+(t3.*t496.*(t105-t465))./2.0);
t4936 = t1838+t2622+t2664+t2703+t2784;
t4944 = -t3967.*(-t2388+t3008+t9.*t868.*(t105-t465).*9.53094055e-4);
t4953 = ITail.*(-t947+t1240.*(t105-t465)+t903.*(t534-t546)).*(-t993+t1535+t1540-t1552+(t3.*t496.*(t105-t465))./2.0);
t4954 = ITail.*(-t1017+(t1240.*(t105-t465))./2.0+(t903.*(t534-t546))./2.0).*(-t1018+t1426+t1431-t1446+t3.*t496.*(t105-t465));
t4971 = -t3967.*(-t1974+t1240.*(t105-t465).*9.53094055e-4+t903.*(t534-t546).*9.53094055e-4);
t4976 = t3967.*(-t1974+t1240.*(t105-t465).*9.53094055e-4+t903.*(t534-t546).*9.53094055e-4);
t5003 = t4207+t4598;
t5021 = ITail.*(-t1355+t1789+(t9.*t868.*(t105-t465))./2.0).*(t1019-t1651+t1702+t3.*t818.*(t105-t465)+t3.*t872.*(t103-t544));
t5032 = ITail.*(-t1262+t1701+t9.*t868.*(t105-t465)).*(t994-t1742+t1790+(t3.*t818.*(t105-t465))./2.0+(t3.*t872.*(t103-t544))./2.0);
t5044 = -t4164.*(-t1974+t1240.*(t105-t465).*9.53094055e-4+t903.*(t534-t546).*9.53094055e-4);
t5053 = -ITail.*t4581.*(-t1017+(t1240.*(t105-t465))./2.0+(t903.*(t534-t546))./2.0);
t5054 = t4164.*(-t1974+t1240.*(t105-t465).*9.53094055e-4+t903.*(t534-t546).*9.53094055e-4);
t5058 = ITail.*t4581.*(-t1017+(t1240.*(t105-t465))./2.0+(t903.*(t534-t546))./2.0);
t5059 = ITail.*(-t1017+(t1240.*(t105-t465))./2.0+(t903.*(t534-t546))./2.0).*(t1019-t1651+t1702+t3.*t818.*(t105-t465)+t3.*t872.*(t103-t544));
t5066 = ITail.*(-t947+t1240.*(t105-t465)+t903.*(t534-t546)).*(t994-t1742+t1790+(t3.*t818.*(t105-t465))./2.0+(t3.*t872.*(t103-t544))./2.0);
t5200 = ITail.*(-t1017+(t1240.*(t105-t465))./2.0+(t903.*(t534-t546))./2.0).*(t1260-t1328-t1427-t1441+t1706+t9.*t870.*(t105-t465));
t5208 = t2052+t2146+t2614+t2683+t2745+t2762;
t5227 = -t4454.*(-t2388+t3008+t9.*t868.*(t105-t465).*9.53094055e-4);
t5265 = -t4454.*(-t1974+t1240.*(t105-t465).*9.53094055e-4+t903.*(t534-t546).*9.53094055e-4);
t5275 = (-t2388+t3008+t9.*t868.*(t105-t465).*9.53094055e-4).*(-t1018+t1426+t1431-t1446+t3.*t496.*(t105-t465));
t5317 = (-t1974+t1240.*(t105-t465).*9.53094055e-4+t903.*(t534-t546).*9.53094055e-4).*(-t1018+t1426+t1431-t1446+t3.*t496.*(t105-t465));
t5399 = (-t2388+t3008+t9.*t868.*(t105-t465).*9.53094055e-4).*(t1019-t1651+t1702+t3.*t818.*(t105-t465)+t3.*t872.*(t103-t544));
t5420 = -t4581.*(-t1974+t1240.*(t105-t465).*9.53094055e-4+t903.*(t534-t546).*9.53094055e-4);
t5424 = t655+t904+t914+t1525+t1857+t1860+t2702+t3237+t3249;
t5431 = t4581.*(-t1974+t1240.*(t105-t465).*9.53094055e-4+t903.*(t534-t546).*9.53094055e-4);
t5438 = (-t1974+t1240.*(t105-t465).*9.53094055e-4+t903.*(t534-t546).*9.53094055e-4).*(t1019-t1651+t1702+t3.*t818.*(t105-t465)+t3.*t872.*(t103-t544));
t5539 = (-t1262+t1701+t9.*t868.*(t105-t465)).*(-t2058+t2688+t2700-t2718+t3.*t496.*(t105-t465).*9.53094055e-4);
t5572 = (-t1974+t1240.*(t105-t465).*9.53094055e-4+t903.*(t534-t546).*9.53094055e-4).*(t1260-t1328-t1427-t1441+t1706+t9.*t870.*(t105-t465));
t5576 = (-t947+t1240.*(t105-t465)+t903.*(t534-t546)).*(-t2058+t2688+t2700-t2718+t3.*t496.*(t105-t465).*9.53094055e-4);
t5674 = (-t1262+t1701+t9.*t868.*(t105-t465)).*(t2059-t2952+t3009+t3.*t818.*(t105-t465).*9.53094055e-4+t3.*t872.*(t103-t544).*9.53094055e-4);
t5706 = (-t947+t1240.*(t105-t465)+t903.*(t534-t546)).*(t2059-t2952+t3009+t3.*t818.*(t105-t465).*9.53094055e-4+t3.*t872.*(t103-t544).*9.53094055e-4);
t5740 = t4716+t4752;
t1339 = -t1291;
t1569 = T_cg_H.*t1510;
t1574 = dphi2.*t1510;
t1575 = dpsi1.*t1510;
t1622 = -t1558;
t1623 = -t1564;
t1630 = -t1578;
t1631 = -t1607;
t1634 = -t1586;
t1662 = t1604./2.0;
t1696 = B_cg_H.*Mb.*t4.*t10.*t1510;
t1697 = B_cg_H.*Mb.*t5.*t9.*t1510;
t1724 = Mb.*t4.*t5.*t1558;
t1763 = t34.*t35.*t1510;
t1780 = B_cg_H.*Mb.*t5.*t30.*t1510;
t1781 = B_cg_H.*Mb.*t5.*t34.*t1510;
t1822 = -t1754;
t1823 = -t1787;
t1848 = t1754./2.0;
t1855 = t1771./2.0;
t1932 = t6.*t381.*t1510;
t1934 = t11.*t381.*t1510;
t1946 = Mb.*t381.*t1558;
t1947 = B_cg_H.*Mb.*t381.*t1510;
t1948 = B_cg_H.*Mb.*t382.*t1510;
t1991 = t496.*t1510;
t2001 = t11.*t420.*t1510;
t2002 = t547.*t1510;
t2010 = Mb.*t421.*t1558;
t2011 = B_cg_H.*Mb.*t420.*t1510;
t2012 = B_cg_H.*Mb.*t421.*t1510;
t2019 = t487.*t1510;
t2032 = t1923./2.0;
t2039 = t1933./2.0;
t2073 = -t1984;
t2080 = -t2036;
t2085 = -t1996;
t2093 = -t2049;
t2101 = t8.*t2014;
t2111 = t559.*t1510;
t2112 = t560.*t1510;
t2115 = t8.*t1992;
t2122 = -t2027;
t2125 = t1987./2.0;
t2133 = t1996./2.0;
t2160 = t2014./2.0;
t2164 = t2022./2.0;
t2166 = t2027./2.0;
t2169 = t2030./2.0;
t2170 = -t2077;
t2175 = -t2137;
t2177 = -t2143;
t2193 = -t2110;
t2194 = -t2163;
t2197 = Mb.*t11.*t15.*t459.*t1510;
t2200 = -t2168;
t2204 = t2077./2.0;
t2210 = t2082./2.0;
t2236 = t2105./2.0;
t2241 = t2110./2.0;
t2270 = -t2184;
t2284 = -t2248;
t2300 = t2184./2.0;
t2313 = t817.*t1510;
t2329 = Mb.*t15.*t675.*t1510;
t2333 = -t2301;
t2355 = t2265./2.0;
t2368 = t903.*t1510;
t2370 = -t2308;
t2374 = -t1510.*(t105-t465);
t2410 = dth2.*t2319;
t2413 = t2308./2.0;
t2444 = t4.*t871.*t1510;
t2448 = -t1510.*(t103-t544);
t2452 = t8.*t872.*t1510;
t2454 = -t2415;
t2457 = -t2418;
t2459 = -t2419;
t2496 = t2364./2.0;
t2498 = t2365./2.0;
t2500 = t2449.*(-1.0./2.0);
t2508 = t1510.*(t105-t465).*(-1.0./2.0);
t2537 = -t1510.*(t197-t537);
t2538 = -t2434;
t2548 = -t2440;
t2549 = -t2441;
t2555 = -t2499;
t2556 = t2449./2.0;
t2559 = -t2507;
t2573 = t2524.*2.0;
t2574 = Mt.*t4.*t10.*t2319;
t2575 = Mt.*t5.*t9.*t2319;
t2578 = t2434./2.0;
t2583 = Mt.*t4.*t5.*t2325;
t2585 = t2439./2.0;
t2593 = t2440./2.0;
t2594 = t2441./2.0;
t2595 = t2442./2.0;
t2602 = t2446./2.0;
t2606 = t1510.*(t103-t544).*(-1.0./2.0);
t2630 = -t2571;
t2642 = t1044.*t1510;
t2644 = -t2580;
t2645 = -t2582;
t2661 = -t2618;
t2672 = Mt.*t5.*t30.*t2319;
t2674 = Mt.*t5.*t34.*t2319;
t2675 = t2631.*2.0;
t2685 = t1510.*(t197-t537).*(-1.0./2.0);
t2726 = t1604.*3.36554e-3;
t2728 = Mb.*t15.*t2524;
t2737 = Mb.*t15.*t977.*t1510;
t2779 = t2641./2.0;
t2796 = Mb.*t15.*t1037.*t1510;
t2798 = -Mb.*t15.*t1510.*(t195-t634);
t2814 = -t2785;
t2829 = t1179.*t1510;
t2848 = -t2822;
t2852 = t1604.*9.52624335e-4;
t2858 = t1604.*3.372816795e-3;
t2861 = Mb.*t15.*t1510.*(t195-t634);
t2868 = t2831.*2.0;
t2893 = -t2850;
t2901 = -t2826;
t2904 = t1240.*t1510;
t2921 = Mt.*t381.*t2319;
t2922 = Mt.*t382.*t2319;
t2925 = t1754.*3.36554e-3;
t2933 = t2826./2.0;
t2934 = t2827./2.0;
t2936 = t1771.*3.36554e-3;
t2937 = Mt.*t381.*t2325;
t2941 = t2831./2.0;
t2986 = Mt.*t420.*t2319;
t2987 = Mt.*t421.*t2319;
t2997 = t2899./2.0;
t2999 = Mt.*t421.*t2325;
t3032 = -t2981;
t3049 = -t3026;
t3071 = t1754.*3.372786875e-3;
t3073 = t1754.*9.53094055e-4;
t3076 = t1771.*3.372786875e-3;
t3080 = t1771.*9.53094055e-4;
t3096 = -t3057;
t3101 = Mt.*t5.*t9.*t2914;
t3123 = t1430.*t1510;
t3139 = t483+t1169+t1278;
t3150 = t1923.*3.36554e-3;
t3156 = t1933.*3.36554e-3;
t3163 = -t3122;
t3178 = -t3142;
t3185 = -t3154;
t3192 = t1505.*t1510;
t3196 = -t3167;
t3198 = -t3169;
t3206 = t482+t623+t624+t1276;
t3211 = t2027.*3.36554e-3;
t3214 = t2030.*3.36554e-3;
t3215 = t1987.*3.36554e-3;
t3225 = t1996.*3.36554e-3;
t3250 = t2014.*3.36554e-3;
t3253 = t2022.*3.36554e-3;
t3255 = Mb.*t5.*t9.*t3082;
t3261 = -t3230;
t3271 = t2077.*3.36554e-3;
t3276 = t2082.*3.36554e-3;
t3283 = t1923.*3.372786875e-3;
t3288 = t3195./2.0;
t3289 = t1923.*9.53094055e-4;
t3300 = t1933.*3.367829185e-3;
t3311 = t2105.*3.36554e-3;
t3312 = t2110.*3.36554e-3;
t3320 = -t3270;
t3326 = -t3279;
t3334 = -t3298;
t3338 = -t3307;
t3340 = -t3309;
t3346 = t2022.*9.52624335e-4;
t3348 = t1933.*8.56645e-6;
t3350 = t2027.*3.372786875e-3;
t3354 = t2030.*3.372786875e-3;
t3356 = t1987.*9.52624335e-4;
t3358 = t2022.*3.372816795e-3;
t3363 = t2027.*9.53094055e-4;
t3365 = t2030.*9.53094055e-4;
t3367 = t1987.*3.372816795e-3;
t3371 = t1996.*3.372786875e-3;
t3374 = t1996.*9.53094055e-4;
t3375 = t2014.*3.367829185e-3;
t3388 = t2184.*3.36554e-3;
t3398 = Mt.*t382.*t2914;
t3400 = -t3345;
t3407 = -t3362;
t3413 = -t3385;
t3414 = -t3389;
t3421 = -t3395;
t3423 = t2105.*3.372816795e-3;
t3424 = t2110.*9.52624335e-4;
t3432 = t2110.*3.372816795e-3;
t3433 = t2077.*9.52624335e-4;
t3439 = t2082.*9.52624335e-4;
t3440 = t2077.*3.372816795e-3;
t3442 = t2082.*3.372816795e-3;
t3445 = t2265.*3.36554e-3;
t3452 = t2014.*8.56645e-6;
t3458 = -t3418;
t3462 = t2105.*9.52624335e-4;
t3465 = -t3422;
t3467 = Mt.*t420.*t2914;
t3472 = -t3427;
t3475 = -t3429;
t3479 = -t3436;
t3480 = -t3437;
t3481 = B_cg_H.*Mb.*t1510.*t1660;
t3485 = -t3446;
t3486 = -t3451;
t3489 = t2308.*3.36554e-3;
t3496 = -t3461;
t3506 = t2184.*9.52624335e-4;
t3509 = -t3490;
t3513 = t2184.*3.372816795e-3;
t3515 = -t3493;
t3517 = -t3498;
t3518 = -t3500;
t3532 = t2364.*3.36554e-3;
t3534 = -t3507;
t3535 = t2365.*3.36554e-3;
t3537 = t2449.*(-3.36554e-3);
t3541 = -t3514;
t3544 = t1510.*(t105-t465).*(-3.36554e-3);
t3550 = -t3525;
t3552 = t2265.*9.52624335e-4;
t3553 = t2265.*3.372816795e-3;
t3554 = Mb.*t382.*t3082;
t3556 = t1510.*(t105-t465).*3.36554e-3;
t3557 = -t3545;
t3558 = -t3546;
t3563 = t2308.*9.53094055e-4;
t3575 = -t3549;
t3582 = t2434.*3.36554e-3;
t3585 = t2439.*3.36554e-3;
t3586 = t2440.*3.36554e-3;
t3587 = t2441.*3.36554e-3;
t3588 = t2442.*3.36554e-3;
t3592 = t2446.*3.36554e-3;
t3593 = t1510.*(t103-t544).*(-3.36554e-3);
t3597 = t2308.*3.372786875e-3;
t3599 = -t3560;
t3600 = -t3561;
t3602 = -t3566;
t3603 = -t3567;
t3604 = -t3568;
t3605 = -t3572;
t3606 = -t3573;
t3607 = -t3576;
t3608 = t2524.*6.73108e-3;
t3613 = -t3584;
t3620 = Mb.*t420.*t3082;
t3623 = t1510.*(t103-t544).*3.36554e-3;
t3625 = -t3598;
t3629 = t2365.*3.372816795e-3;
t3631 = t1510.*(t105-t465).*(-3.372786875e-3);
t3633 = t2449.*(-9.53094055e-4);
t3640 = t1510.*(t105-t465).*(-9.53094055e-4);
t3645 = t2449.*(-3.367829185e-3);
t3648 = t1510.*(t105-t465).*(-3.367829185e-3);
t3653 = t1510.*(t197-t537).*(-3.36554e-3);
t3654 = -t3612;
t3660 = t2364.*3.372786875e-3;
t3661 = t2365.*9.52624335e-4;
t3664 = t2449.*(-3.372786875e-3);
t3667 = t2364.*9.53094055e-4;
t3668 = -t3627;
t3669 = t2449.*9.53094055e-4;
t3673 = -t3642;
t3674 = t2631.*6.73108e-3;
t3675 = t1510.*(t105-t465).*3.367829185e-3;
t3676 = -t3649;
t3688 = -t3659;
t3689 = -t3662;
t3692 = -t3628;
t3694 = t2446.*3.372816795e-3;
t3695 = t1510.*(t103-t544).*(-9.53094055e-4);
t3707 = t1510.*(t103-t544).*(-3.367829185e-3);
t3711 = t2641.*3.36554e-3;
t3714 = t2434.*9.52624335e-4;
t3718 = t2449.*(-8.56645e-6);
t3720 = t2434.*3.372816795e-3;
t3723 = t2439.*9.52624335e-4;
t3725 = t1510.*(t105-t465).*(-8.56645e-6);
t3727 = t2440.*9.52624335e-4;
t3728 = t2441.*9.52624335e-4;
t3729 = t2442.*9.52624335e-4;
t3731 = t2439.*3.372816795e-3;
t3733 = t2446.*9.52624335e-4;
t3734 = t2440.*3.372816795e-3;
t3735 = t2441.*3.372816795e-3;
t3736 = t2442.*3.372816795e-3;
t3737 = t1510.*(t103-t544).*(-3.372786875e-3);
t3742 = -t3696;
t3745 = -t3703;
t3747 = t1510.*(t103-t544).*3.367829185e-3;
t3753 = -t3716;
t3754 = t2449.*8.56645e-6;
t3762 = -t3722;
t3770 = t466+t751+t879+t1564;
t3773 = t2524.*1.90524867e-3;
t3776 = t2524.*6.74563359e-3;
t3778 = t1510.*(t197-t537).*(-9.52624335e-4);
t3785 = t1510.*(t197-t537).*(-3.372816795e-3);
t3786 = t1510.*(t103-t544).*(-8.56645e-6);
t3796 = -t3782;
t3799 = -t3788;
t3801 = t2831.*6.73108e-3;
t3802 = dphi2.*t3780;
t3803 = t2631.*1.90524867e-3;
t3806 = t2631.*6.74563359e-3;
C = ft_8({B_cg_H,ITail,Mb,Mm,Mt,T_cg_H,dphi1,dphi2,dpsi1,dth1,dth2,dx,dy,dz,t10,t1003,t1004,t1005,t1006,t1007,t1008,t1009,t1010,t1011,t1012,t1013,t1014,t1015,t1016,t1017,t1018,t1019,t1020,t1023,t1026,t1029,t103,t1031,t1037,t1041,t1042,t1044,t1045,t1046,t1047,t1049,t105,t1050,t1051,t1052,t1053,t1054,t1055,t1056,t1057,t1059,t1060,t1061,t1063,t1064,t1065,t1067,t1068,t1071,t1072,t1073,t1074,t1075,t1076,t1077,t1078,t1079,t1082,t1084,t1086,t1088,t1097,t1099,t11,t1102,t1107,t1108,t1113,t1114,t1115,t1116,t1117,t1118,t1119,t1120,t1121,t1122,t1123,t1124,t1125,t1127,t1128,t1129,t1131,t1132,t1133,t1134,t1135,t1136,t1137,t1138,t1139,t1140,t1141,t1142,t1143,t1144,t1146,t1147,t1149,t1152,t1153,t1154,t1155,t1156,t1157,t1158,t1159,t1160,t1161,t1162,t1163,t1164,t1166,t1167,t1168,t1169,t1170,t1171,t1172,t1173,t1174,t1176,t1177,t1178,t1179,t1181,t1182,t1183,t1184,t1185,t1186,t1187,t1188,t1189,t1190,t1191,t1192,t1193,t1194,t1195,t1196,t1197,t1199,t120,t1200,t1201,t1202,t1203,t1205,t1206,t1211,t1212,t1213,t1214,t1215,t1220,t1221,t1223,t1224,t1225,t1226,t1228,t1229,t123,t1230,t1231,t1232,t1234,t1236,t1237,t1240,t1242,t1243,t1244,t1245,t1246,t1247,t1248,t1250,t1251,t1252,t1253,t1255,t1256,t1257,t1260,t1261,t1262,t1263,t1264,t1265,t1268,t1271,t1272,t1275,t1280,t1282,t1283,t1285,t1286,t1288,t1291,t1293,t1295,t1296,t1297,t1299,t130,t1301,t1302,t1303,t1304,t1305,t1306,t1307,t1308,t1309,t1311,t1312,t1313,t1319,t1320,t1322,t1323,t1324,t1325,t1328,t1329,t1331,t1332,t1334,t1337,t1338,t1339,t134,t1340,t1341,t1343,t1344,t1345,t1348,t1349,t1352,t1354,t1355,t1356,t1357,t1358,t1360,t1361,t1362,t1365,t1366,t1367,t1368,t1370,t1371,t1373,t1374,t1378,t1379,t1380,t1381,t1382,t1383,t1384,t1386,t1388,t1389,t1391,t1393,t1394,t1395,t1396,t1397,t1399,t1402,t1403,t1405,t1406,t1407,t1408,t1409,t1410,t1412,t1413,t1414,t1415,t1416,t1418,t1419,t1421,t1422,t1423,t1426,t1427,t1430,t1431,t1433,t1435,t1437,t1438,t1439,t144,t1440,t1441,t1442,t1443,t1444,t1445,t1446,t1448,t1450,t1451,t1453,t1455,t1456,t1457,t1458,t1459,t1460,t1461,t1463,t1465,t1466,t1467,t1468,t1469,t1470,t1473,t1476,t1477,t1478,t1479,t1480,t1481,t1482,t1483,t1484,t1486,t1487,t1488,t1489,t1491,t1492,t1493,t1495,t1496,t1497,t1498,t15,t1500,t1505,t1506,t1508,t1509,t1510,t1512,t1513,t1515,t1516,t1517,t1518,t1519,t1520,t1521,t1522,t1523,t1525,t1526,t1527,t1528,t1529,t1531,t1532,t1535,t1537,t1539,t1540,t1542,t1543,t1544,t1546,t1547,t1548,t1549,t1550,t1551,t1552,t1553,t1555,t1558,t1559,t1560,t1561,t1562,t1563,t1565,t1566,t1567,t1568,t1569,t1570,t1571,t1574,t1575,t1576,t1577,t1578,t1579,t1580,t1581,t1582,t1583,t1584,t1585,t1586,t1587,t1589,t1590,t1591,t1592,t1593,t1594,t1595,t1596,t1597,t1598,t1599,t160,t1601,t1602,t1604,t1605,t1606,t1609,t161,t1610,t1612,t1614,t1615,t1616,t1617,t1618,t1619,t162,t1620,t1621,t1622,t1623,t1624,t1625,t1626,t1627,t1628,t1630,t1631,t1632,t1633,t1634,t1635,t1636,t1637,t1638,t1639,t1640,t1641,t1642,t1643,t1644,t1645,t1646,t1649,t1651,t1652,t1653,t1654,t1655,t1656,t1657,t1658,t1659,t1660,t1661,t1662,t1663,t1664,t1665,t1666,t1667,t1668,t1669,t1671,t1672,t1674,t1675,t1676,t1677,t1678,t1679,t1680,t1681,t1682,t1683,t1684,t1685,t1686,t1687,t1688,t1689,t1690,t1691,t1692,t1693,t1694,t1695,t1696,t1697,t1698,t1699,t1700,t1701,t1702,t1703,t1704,t1705,t1706,t1711,t1715,t1716,t1718,t1719,t1720,t1721,t1722,t1723,t1725,t1726,t1727,t1729,t1730,t1731,t1732,t1733,t1734,t1735,t1736,t1737,t1739,t1740,t1741,t1742,t1743,t1744,t1745,t1746,t1747,t1748,t1749,t1750,t1751,t1753,t1755,t1756,t1758,t1759,t1761,t1762,t1763,t1764,t1765,t1769,t1770,t1771,t1774,t1777,t1778,t1779,t1780,t1781,t1783,t1784,t1785,t1786,t1787,t1788,t1789,t1790,t1791,t1792,t1796,t1798,t1799,t1800,t1801,t1802,t1803,t1806,t1809,t1810,t1811,t1812,t1813,t1814,t1815,t1816,t1817,t1819,t1820,t1821,t1822,t1823,t1824,t1825,t1826,t1827,t1828,t1829,t1830,t1831,t1832,t1833,t1834,t1835,t1836,t1839,t1841,t1842,t1843,t1844,t1845,t1846,t1847,t1848,t1849,t1851,t1852,t1855,t1856,t1857,t1858,t1859,t1860,t1862,t1863,t1864,t1865,t1866,t1867,t1870,t1871,t1872,t1873,t1874,t1875,t1877,t1878,t1880,t1881,t1882,t1883,t1884,t1885,t1887,t1888,t1890,t1891,t1893,t1894,t1895,t1896,t1898,t1899,t1900,t1902,t1904,t1905,t1906,t1907,t1908,t1909,t1910,t1911,t1912,t1913,t1914,t1915,t1916,t1917,t1918,t1919,t1920,t1921,t1922,t1923,t1924,t1926,t1928,t1929,t1930,t1931,t1932,t1933,t1934,t1935,t1937,t1938,t1939,t1940,t1941,t1942,t1943,t1945,t1946,t1947,t1948,t1949,t195,t1950,t1951,t1952,t1953,t1955,t1956,t1957,t1959,t1960,t1961,t1962,t1963,t1964,t1965,t1966,t1967,t1968,t1969,t197,t1970,t1971,t1973,t1974,t1975,t1976,t1977,t1978,t1979,t1980,t1981,t1982,t1983,t1984,t1985,t1986,t1987,t1988,t1989,t1990,t1991,t1992,t1993,t1994,t1995,t1998,t1999,t2,t2000,t2001,t2002,t2004,t2005,t2006,t2007,t2008,t2009,t2010,t2011,t2012,t2014,t2015,t2016,t2017,t2018,t2019,t2020,t2023,t2024,t2025,t2026,t2028,t2030,t2032,t2033,t2035,t2037,t2039,t2041,t2042,t2043,t2045,t2046,t2047,t2048,t2049,t2050,t2053,t2057,t2058,t2059,t2060,t2061,t2062,t2063,t2064,t2065,t2066,t2067,t2068,t2069,t2070,t2072,t2073,t2074,t2075,t2076,t2078,t2079,t2080,t2081,t2082,t2083,t2084,t2085,t2087,t2088,t2090,t2091,t2092,t2093,t2094,t2095,t2096,t2097,t2098,t2099,t2100,t2101,t2102,t2103,t2104,t2105,t2106,t2108,t2109,t2110,t2111,t2112,t2113,t2114,t2115,t2116,t2117,t2118,t2119,t2120,t2121,t2122,t2123,t2124,t2125,t2126,t2127,t2129,t2130,t2131,t2132,t2133,t2134,t2135,t2136,t2137,t214,t2141,t2142,t2143,t2144,t2147,t2148,t2149,t2150,t2151,t2152,t2153,t2154,t2155,t2156,t2157,t2158,t2160,t2161,t2164,t2165,t2166,t2167,t2169,t2170,t2171,t2172,t2174,t2175,t2176,t2177,t2178,t2179,t2181,t2182,t2183,t2186,t2187,t2188,t2189,t2190,t2191,t2192,t2193,t2194,t2196,t2197,t2199,t2200,t2201,t2202,t2203,t2204,t2205,t2206,t2208,t2209,t2210,t2211,t2212,t2213,t2214,t2215,t2216,t2217,t2218,t2219,t2220,t2221,t2222,t2223,t2224,t2225,t2227,t2228,t2229,t2230,t2232,t2233,t2235,t2236,t2237,t2238,t2239,t2240,t2241,t2242,t2245,t2246,t2247,t2248,t2249,t2251,t2252,t2253,t2254,t2255,t2257,t2258,t2259,t2260,t2262,t2263,t2265,t2267,t2268,t2269,t2270,t2271,t2272,t2274,t2276,t2277,t2281,t2284,t2285,t2286,t2287,t2288,t2289,t2290,t2292,t2293,t2294,t2296,t2298,t2299,t2300,t2303,t2304,t2305,t2307,t2308,t2309,t2312,t2313,t2314,t2316,t2317,t2318,t2319,t2320,t2321,t2322,t2323,t2324,t2325,t2327,t2328,t2329,t2330,t2331,t2333,t2334,t2335,t2336,t2338,t2339,t2340,t2341,t2342,t2343,t2344,t2345,t2346,t2347,t2348,t2349,t2350,t2351,t2352,t2354,t2355,t2356,t2358,t2360,t2361,t2362,t2363,t2364,t2365,t2368,t2369,t2370,t2371,t2373,t2374,t2375,t2376,t2377,t2378,t2380,t2381,t2382,t2385,t2386,t2387,t2388,t2389,t2390,t2392,t2396,t2397,t2399,t24,t2400,t2401,t2403,t2404,t2406,t2407,t2408,t2409,t2410,t2411,t2412,t2413,t2414,t2417,t2419,t2420,t2422,t2423,t2425,t2426,t2427,t2428,t2429,t2430,t2431,t2432,t2433,t2434,t2435,t2436,t2437,t2438,t2439,t2442,t2443,t2444,t2445,t2446,t2447,t2448,t2449,t2452,t2453,t2454,t2455,t2457,t2458,t2459,t2460,t2461,t2462,t2463,t2464,t2465,t2466,t2467,t2468,t2469,t2470,t2471,t2472,t2474,t2476,t2479,t2480,t2483,t2484,t2485,t2486,t2487,t2488,t2489,t2492,t2495,t2496,t2498,t25,t2502,t2503,t2504,t2505,t2506,t2508,t2509,t2511,t2512,t2513,t2514,t2515,t2516,t2518,t2519,t2520,t2521,t2522,t2523,t2524,t2525,t2526,t2527,t2528,t2529,t2530,t2531,t2532,t2533,t2534,t2535,t2536,t2537,t2538,t2539,t2541,t2542,t2543,t2544,t2545,t2546,t2547,t2548,t2549,t2550,t2551,t2552,t2555,t2556,t2559,t2560,t2561,t2562,t2563,t2564,t2565,t2566,t2567,t2568,t2569,t2570,t2571,t2573,t2574,t2575,t2576,t2577,t2578,t2579,t2581,t2582,t2583,t2584,t2585,t2587,t2588,t2589,t259,t2590,t2591,t2593,t2594,t2595,t2596,t2597,t2598,t2599,t26,t260,t2600,t2602,t2605,t2606,t2607,t2610,t2611,t2612,t2613,t2615,t2616,t2617,t2619,t2620,t2621,t2623,t2624,t2627,t2629,t2630,t2631,t2632,t2634,t2635,t2636,t2637,t2638,t2640,t2641,t2642,t2643,t2644,t2645,t2646,t2647,t2648,t2649,t2650,t2654,t2656,t2657,t2658,t2660,t2661,t2662,t2663,t2665,t2666,t2667,t2668,t2669,t2671,t2672,t2673,t2674,t2675,t2677,t2678,t2679,t2681,t2682,t2684,t2685,t2688,t2689,t2691,t2692,t2695,t2696,t2698,t2699,t27,t2700,t2704,t2705,t2706,t2707,t2708,t2710,t2711,t2712,t2714,t2715,t2717,t2718,t2722,t2723,t2725,t2726,t2727,t2728,t2730,t2731,t2732,t2733,t2735,t2736,t2737,t2738,t2739,t2740,t2742,t2743,t2744,t2746,t2747,t2748,t2749,t2750,t2751,t2752,t2754,t2755,t2756,t2758,t2759,t276,t2760,t2761,t2763,t2764,t2765,t2766,t2768,t2769,t277,t2770,t2771,t2772,t2774,t2775,t2776,t2778,t2779,t2781,t2782,t2783,t2785,t2786,t2787,t2788,t2790,t2791,t2792,t2793,t2795,t2796,t2797,t2798,t2799,t28,t2800,t2802,t2803,t2804,t2806,t2807,t2811,t2813,t2814,t2816,t2817,t2818,t2819,t2821,t2823,t2824,t2825,t2826,t2827,t2828,t2829,t283,t2830,t2831,t2832,t2833,t2834,t2835,t2836,t2837,t2838,t2839,t284,t2841,t2842,t2843,t2844,t2845,t2846,t2847,t2848,t2849,t285,t2851,t2852,t2853,t2857,t2858,t2859,t286,t2860,t2861,t2862,t2864,t2865,t2866,t2867,t2868,t2869,t287,t2870,t2871,t2872,t2874,t2875,t2876,t2877,t2878,t2879,t288,t2880,t2881,t2882,t2883,t2884,t2885,t2886,t2887,t2889,t289,t2890,t2892,t2893,t2895,t2896,t2897,t2898,t2899,t290,t2900,t2901,t2902,t2903,t2904,t2906,t2907,t2909,t291,t2912,t2913,t2914,t2915,t2916,t2917,t2918,t2919,t292,t2920,t2921,t2922,t2923,t2924,t2925,t2926,t2927,t2928,t2929,t293,t2932,t2933,t2934,t2935,t2936,t2937,t2938,t294,t2940,t2941,t2942,t2943,t2944,t2945,t2946,t2947,t2949,t2950,t2951,t2952,t2954,t2955,t2956,t2957,t2959,t2960,t2961,t2962,t2963,t2964,t2966,t2967,t2969,t2972,t2975,t2976,t2977,t2978,t2979,t2981,t2982,t2985,t2986,t2987,t2988,t2989,t2992,t2994,t2995,t2996,t2997,t2998,t2999,t3,t30,t3003,t3004,t3006,t3007,t3008,t3009,t3010,t3011,t3012,t3016,t3017,t3019,t3020,t3022,t3023,t3027,t3030,t3031,t3032,t3033,t3034,t3035,t3036,t3037,t3038,t3039,t304,t3041,t3042,t3043,t3044,t3045,t3046,t3047,t3049,t3050,t3051,t3054,t3059,t3060,t3061,t3062,t3063,t3064,t3065,t3066,t3069,t3070,t3071,t3072,t3073,t3074,t3075,t3076,t3077,t3078,t3080,t3081,t3082,t3083,t3084,t3085,t3087,t3089,t3090,t3091,t3092,t3093,t3094,t3095,t3096,t3097,t3098,t3099,t3100,t3101,t3102,t3105,t3106,t3107,t3108,t3109,t3110,t3112,t3113,t3114,t3115,t3117,t3119,t3122,t3123,t3124,t3127,t3128,t3130,t3131,t3132,t3133,t3134,t3135,t3136,t3138,t3139,t3143,t3145,t3146,t3147,t3149,t3150,t3151,t3153,t3156,t3157,t3158,t3160,t3162,t3163,t3164,t3165,t3166,t3167,t3169,t3170,t3171,t3173,t3174,t3175,t3176,t3177,t3178,t3179,t3180,t3181,t3184,t3185,t3186,t3187,t3189,t3192,t3195,t3196,t3197,t3198,t3199,t3200,t3203,t3204,t3206,t3207,t3210,t3211,t3212,t3213,t3214,t3215,t3216,t3217,t3218,t3220,t3221,t3222,t3223,t3224,t3225,t3226,t3228,t3229,t3230,t3233,t3235,t3236,t3238,t3239,t3240,t3241,t3243,t3244,t3245,t3246,t3247,t3248,t3250,t3252,t3253,t3255,t3256,t3260,t3261,t3263,t3265,t3266,t3270,t3271,t3272,t3273,t3274,t3275,t3276,t3277,t3278,t3279,t3280,t3281,t3282,t3283,t3284,t3285,t3286,t3287,t3288,t3289,t3290,t3291,t3294,t3295,t3296,t33,t3300,t3301,t3303,t3304,t3305,t3306,t3307,t3311,t3312,t3315,t3317,t3319,t3320,t3321,t3322,t3323,t3325,t3326,t3330,t3331,t3332,t3333,t3334,t3337,t3338,t3339,t3340,t3341,t3346,t3348,t3350,t3351,t3353,t3354,t3356,t3357,t3358,t3359,t3360,t3361,t3363,t3364,t3365,t3366,t3367,t3368,t3369,t3370,t3371,t3372,t3373,t3374,t3375,t3376,t3378,t3379,t3380,t3381,t3384,t3385,t3388,t3390,t3391,t3392,t3393,t3397,t3398,t3399,t34,t3400,t3403,t3407,t3412,t3413,t3414,t3415,t3416,t3419,t3420,t3421,t3423,t3424,t3425,t3426,t3427,t3429,t3432,t3433,t3434,t3437,t3438,t3439,t3440,t3441,t3442,t3445,t3446,t3447,t3448,t3449,t3450,t3452,t3453,t3454,t3457,t3458,t3459,t3460,t3462,t3465,t3467,t3468,t3469,t3471,t3472,t3474,t3475,t3478,t3479,t3480,t3481,t3483,t3484,t3485,t3486,t3487,t3488,t3489,t3490,t3492,t3495,t3496,t3499,t3500,t3501,t3502,t3504,t3506,t3509,t3512,t3513,t3515,t3516,t3517,t3518,t3520,t3521,t3522,t3523,t3524,t3527,t3528,t3529,t3530,t3531,t3532,t3534,t3535,t3536,t3537,t3539,t3541,t3542,t3543,t3544,t3545,t3547,t3548,t3550,t3551,t3552,t3553,t3554,t3556,t3557,t3558,t3559,t3562,t3563,t3564,t3565,t3569,t3570,t3571,t3574,t3575,t3576,t3579,t3581,t3582,t3583,t3584,t3585,t3586,t3587,t3588,t3590,t3592,t3593,t3595,t3596,t3597,t3598,t3599,t3600,t3602,t3603,t3604,t3605,t3606,t3607,t3608,t3609,t3611,t3613,t3614,t3617,t3619,t3620,t3621,t3623,t3625,t3626,t3627,t3628,t3629,t3630,t3631,t3632,t3635,t3636,t3637,t3638,t3639,t3640,t3641,t3643,t3644,t3645,t3647,t3648,t3649,t3651,t3652,t3653,t3654,t3655,t3656,t3657,t3659,t3660,t3661,t3663,t3664,t3666,t3667,t3668,t3669,t3671,t3672,t3673,t3674,t3675,t3676,t3677,t3678,t3679,t3680,t3683,t3684,t3686,t3687,t3688,t3689,t3692,t3694,t3695,t3698,t3699,t3700,t3701,t3702,t3704,t3706,t3708,t3709,t3710,t3711,t3713,t3714,t3716,t3717,t3720,t3721,t3722,t3723,t3724,t3725,t3726,t3727,t3728,t3729,t3730,t3731,t3733,t3734,t3735,t3736,t3737,t3739,t3742,t3744,t3745,t3746,t3747,t3749,t375,t3750,t3752,t3753,t3754,t3759,t376,t3761,t3762,t3768,t3769,t377,t3770,t3771,t3772,t3773,t3775,t3776,t3777,t3778,t3779,t3780,t3781,t3783,t3784,t3785,t3786,t3787,t3789,t3790,t3791,t3792,t3793,t3794,t3795,t3796,t3799,t38,t3801,t3802,t3803,t3804,t3805,t3806,t3807,t3808,t381,t3814,t3815,t3819,t382,t3822,t3823,t3828,t383,t3832,t3836,t3838,t3842,t3843,t3844,t3845,t3846,t3847,t3851,t3854,t3855,t3858,t3859,t3862,t3866,t3871,t3873,t3877,t3880,t3882,t3883,t3889,t3898,t3899,t390,t3900,t3902,t3906,t3907,t3908,t3909,t3910,t3913,t3915,t3916,t3918,t3919,t3924,t3926,t3928,t3929,t3930,t3931,t3932,t3933,t3936,t3937,t3939,t394,t3940,t3942,t3944,t3950,t3952,t3955,t3956,t3957,t3959,t3960,t3961,t3962,t3964,t3965,t3967,t3969,t3971,t3974,t3976,t3981,t3982,t3983,t3985,t3993,t3994,t3995,t3996,t3998,t3999,t4,t4000,t4002,t4003,t4005,t4008,t401,t4012,t4014,t4023,t4024,t4028,t4029,t4033,t4035,t4036,t4038,t4042,t4045,t4046,t4047,t4048,t4049,t4051,t4052,t4053,t4054,t4055,t4056,t4058,t4059,t4060,t4061,t4064,t4067,t4068,t4069,t4070,t4071,t4072,t4073,t4074,t4075,t4076,t4078,t4079,t4081,t4086,t4087,t4089,t4090,t4092,t4093,t4094,t4095,t4097,t4098,t4099,t41,t410,t4100,t4101,t4104,t4109,t411,t4112,t4118,t4119,t412,t4121,t4122,t4123,t4124,t4125,t4126,t413,t4130,t4134,t4135,t4137,t414,t4140,t4141,t4143,t4146,t415,t4153,t4155,t4156,t4157,t4158,t4159,t4164,t4165,t4169,t4171,t4174,t4175,t4182,t4188,t4189,t4190,t4196,t4197,t4198,t420,t4203,t421,t4210,t4211,t4212,t4213,t4217,t4218,t4222,t4224,t4225,t4226,t4227,t4231,t4232,t4234,t4236,t4237,t4240,t4241,t4246,t4247,t425,t4253,t4256,t4269,t4270,t4274,t4276,t4282,t4286,t4290,t4295,t4298,t430,t4300,t4301,t4304,t4306,t431,t4312,t4316,t4323,t4324,t4325,t4326,t433,t4330,t4332,t4339,t4342,t4348,t4349,t4354,t4355,t4356,t4358,t436,t4364,t4367,t4368,t4371,t4393,t4395,t44,t4406,t4418,t4420,t4421,t4424,t4432,t445,t4453,t4454,t4457,t4458,t4464,t4475,t4477,t4479,t4481,t4487,t4490,t4492,t4495,t4496,t4497,t450,t4506,t451,t4512,t4525,t4538,t4545,t4549,t4551,t4581,t459,t4597,t4598,t46,t4602,t4603,t4628,t4646,t4649,t465,t4659,t4665,t4695,t4711,t4732,t4739,t4740,t4752,t4789,t4796,t48,t482,t483,t484,t485,t487,t4873,t488,t49,t4909,t491,t4925,t4931,t4932,t4936,t4944,t4953,t4954,t496,t4976,t4995,t5,t50,t501,t502,t5021,t5032,t504,t5053,t5054,t5058,t5059,t5066,t51,t514,t519,t5200,t5208,t5227,t523,t524,t5265,t527,t5275,t530,t5317,t534,t537,t539,t5399,t54,t541,t542,t5420,t5424,t5431,t5438,t544,t546,t55,t550,t553,t5539,t557,t5572,t5576,t558,t56,t5674,t57,t5706,t573,t574,t575,t587,t59,t595,t603,t61,t614,t623,t624,t627,t628,t629,t632,t634,t641,t644,t65,t650,t651,t655,t657,t664,t665,t666,t667,t668,t669,t674,t675,t68,t693,t699,t7,t71,t720,t721,t724,t73,t731,t732,t735,t736,t741,t744,t746,t749,t752,t753,t754,t755,t756,t757,t759,t760,t761,t762,t764,t765,t769,t772,t774,t776,t778,t779,t792,t795,t797,t799,t8,t802,t803,t806,t811,t817,t818,t820,t821,t823,t824,t828,t831,t834,t837,t838,t839,t841,t842,t843,t844,t845,t846,t847,t848,t850,t851,t852,t853,t854,t855,t864,t865,t867,t868,t870,t871,t872,t874,t875,t876,t877,t885,t886,t888,t889,t890,t891,t892,t893,t896,t897,t898,t9,t901,t902,t903,t904,t906,t907,t908,t909,t912,t914,t915,t916,t918,t923,t924,t925,t926,t927,t928,t934,t947,t949,t950,t951,t952,t953,t954,t955,t957,t964,t965,t970,t972,t977,t979,t980,t983,t985,t987,t991,t992,t993,t994,t995,t996});
end
function C = ft_8(ct)
B_cg_H = ct{1};
ITail = ct{2};
Mb = ct{3};
Mm = ct{4};
Mt = ct{5};
T_cg_H = ct{6};
dphi1 = ct{7};
dphi2 = ct{8};
dpsi1 = ct{9};
dth1 = ct{10};
dth2 = ct{11};
dx = ct{12};
dy = ct{13};
dz = ct{14};
t10 = ct{15};
t1003 = ct{16};
t1004 = ct{17};
t1005 = ct{18};
t1006 = ct{19};
t1007 = ct{20};
t1008 = ct{21};
t1009 = ct{22};
t1010 = ct{23};
t1011 = ct{24};
t1012 = ct{25};
t1013 = ct{26};
t1014 = ct{27};
t1015 = ct{28};
t1016 = ct{29};
t1017 = ct{30};
t1018 = ct{31};
t1019 = ct{32};
t1020 = ct{33};
t1023 = ct{34};
t1026 = ct{35};
t1029 = ct{36};
t103 = ct{37};
t1031 = ct{38};
t1037 = ct{39};
t1041 = ct{40};
t1042 = ct{41};
t1044 = ct{42};
t1045 = ct{43};
t1046 = ct{44};
t1047 = ct{45};
t1049 = ct{46};
t105 = ct{47};
t1050 = ct{48};
t1051 = ct{49};
t1052 = ct{50};
t1053 = ct{51};
t1054 = ct{52};
t1055 = ct{53};
t1056 = ct{54};
t1057 = ct{55};
t1059 = ct{56};
t1060 = ct{57};
t1061 = ct{58};
t1063 = ct{59};
t1064 = ct{60};
t1065 = ct{61};
t1067 = ct{62};
t1068 = ct{63};
t1071 = ct{64};
t1072 = ct{65};
t1073 = ct{66};
t1074 = ct{67};
t1075 = ct{68};
t1076 = ct{69};
t1077 = ct{70};
t1078 = ct{71};
t1079 = ct{72};
t1082 = ct{73};
t1084 = ct{74};
t1086 = ct{75};
t1088 = ct{76};
t1097 = ct{77};
t1099 = ct{78};
t11 = ct{79};
t1102 = ct{80};
t1107 = ct{81};
t1108 = ct{82};
t1113 = ct{83};
t1114 = ct{84};
t1115 = ct{85};
t1116 = ct{86};
t1117 = ct{87};
t1118 = ct{88};
t1119 = ct{89};
t1120 = ct{90};
t1121 = ct{91};
t1122 = ct{92};
t1123 = ct{93};
t1124 = ct{94};
t1125 = ct{95};
t1127 = ct{96};
t1128 = ct{97};
t1129 = ct{98};
t1131 = ct{99};
t1132 = ct{100};
t1133 = ct{101};
t1134 = ct{102};
t1135 = ct{103};
t1136 = ct{104};
t1137 = ct{105};
t1138 = ct{106};
t1139 = ct{107};
t1140 = ct{108};
t1141 = ct{109};
t1142 = ct{110};
t1143 = ct{111};
t1144 = ct{112};
t1146 = ct{113};
t1147 = ct{114};
t1149 = ct{115};
t1152 = ct{116};
t1153 = ct{117};
t1154 = ct{118};
t1155 = ct{119};
t1156 = ct{120};
t1157 = ct{121};
t1158 = ct{122};
t1159 = ct{123};
t1160 = ct{124};
t1161 = ct{125};
t1162 = ct{126};
t1163 = ct{127};
t1164 = ct{128};
t1166 = ct{129};
t1167 = ct{130};
t1168 = ct{131};
t1169 = ct{132};
t1170 = ct{133};
t1171 = ct{134};
t1172 = ct{135};
t1173 = ct{136};
t1174 = ct{137};
t1176 = ct{138};
t1177 = ct{139};
t1178 = ct{140};
t1179 = ct{141};
t1181 = ct{142};
t1182 = ct{143};
t1183 = ct{144};
t1184 = ct{145};
t1185 = ct{146};
t1186 = ct{147};
t1187 = ct{148};
t1188 = ct{149};
t1189 = ct{150};
t1190 = ct{151};
t1191 = ct{152};
t1192 = ct{153};
t1193 = ct{154};
t1194 = ct{155};
t1195 = ct{156};
t1196 = ct{157};
t1197 = ct{158};
t1199 = ct{159};
t120 = ct{160};
t1200 = ct{161};
t1201 = ct{162};
t1202 = ct{163};
t1203 = ct{164};
t1205 = ct{165};
t1206 = ct{166};
t1211 = ct{167};
t1212 = ct{168};
t1213 = ct{169};
t1214 = ct{170};
t1215 = ct{171};
t1220 = ct{172};
t1221 = ct{173};
t1223 = ct{174};
t1224 = ct{175};
t1225 = ct{176};
t1226 = ct{177};
t1228 = ct{178};
t1229 = ct{179};
t123 = ct{180};
t1230 = ct{181};
t1231 = ct{182};
t1232 = ct{183};
t1234 = ct{184};
t1236 = ct{185};
t1237 = ct{186};
t1240 = ct{187};
t1242 = ct{188};
t1243 = ct{189};
t1244 = ct{190};
t1245 = ct{191};
t1246 = ct{192};
t1247 = ct{193};
t1248 = ct{194};
t1250 = ct{195};
t1251 = ct{196};
t1252 = ct{197};
t1253 = ct{198};
t1255 = ct{199};
t1256 = ct{200};
t1257 = ct{201};
t1260 = ct{202};
t1261 = ct{203};
t1262 = ct{204};
t1263 = ct{205};
t1264 = ct{206};
t1265 = ct{207};
t1268 = ct{208};
t1271 = ct{209};
t1272 = ct{210};
t1275 = ct{211};
t1280 = ct{212};
t1282 = ct{213};
t1283 = ct{214};
t1285 = ct{215};
t1286 = ct{216};
t1288 = ct{217};
t1291 = ct{218};
t1293 = ct{219};
t1295 = ct{220};
t1296 = ct{221};
t1297 = ct{222};
t1299 = ct{223};
t130 = ct{224};
t1301 = ct{225};
t1302 = ct{226};
t1303 = ct{227};
t1304 = ct{228};
t1305 = ct{229};
t1306 = ct{230};
t1307 = ct{231};
t1308 = ct{232};
t1309 = ct{233};
t1311 = ct{234};
t1312 = ct{235};
t1313 = ct{236};
t1319 = ct{237};
t1320 = ct{238};
t1322 = ct{239};
t1323 = ct{240};
t1324 = ct{241};
t1325 = ct{242};
t1328 = ct{243};
t1329 = ct{244};
t1331 = ct{245};
t1332 = ct{246};
t1334 = ct{247};
t1337 = ct{248};
t1338 = ct{249};
t1339 = ct{250};
t134 = ct{251};
t1340 = ct{252};
t1341 = ct{253};
t1343 = ct{254};
t1344 = ct{255};
t1345 = ct{256};
t1348 = ct{257};
t1349 = ct{258};
t1352 = ct{259};
t1354 = ct{260};
t1355 = ct{261};
t1356 = ct{262};
t1357 = ct{263};
t1358 = ct{264};
t1360 = ct{265};
t1361 = ct{266};
t1362 = ct{267};
t1365 = ct{268};
t1366 = ct{269};
t1367 = ct{270};
t1368 = ct{271};
t1370 = ct{272};
t1371 = ct{273};
t1373 = ct{274};
t1374 = ct{275};
t1378 = ct{276};
t1379 = ct{277};
t1380 = ct{278};
t1381 = ct{279};
t1382 = ct{280};
t1383 = ct{281};
t1384 = ct{282};
t1386 = ct{283};
t1388 = ct{284};
t1389 = ct{285};
t1391 = ct{286};
t1393 = ct{287};
t1394 = ct{288};
t1395 = ct{289};
t1396 = ct{290};
t1397 = ct{291};
t1399 = ct{292};
t1402 = ct{293};
t1403 = ct{294};
t1405 = ct{295};
t1406 = ct{296};
t1407 = ct{297};
t1408 = ct{298};
t1409 = ct{299};
t1410 = ct{300};
t1412 = ct{301};
t1413 = ct{302};
t1414 = ct{303};
t1415 = ct{304};
t1416 = ct{305};
t1418 = ct{306};
t1419 = ct{307};
t1421 = ct{308};
t1422 = ct{309};
t1423 = ct{310};
t1426 = ct{311};
t1427 = ct{312};
t1430 = ct{313};
t1431 = ct{314};
t1433 = ct{315};
t1435 = ct{316};
t1437 = ct{317};
t1438 = ct{318};
t1439 = ct{319};
t144 = ct{320};
t1440 = ct{321};
t1441 = ct{322};
t1442 = ct{323};
t1443 = ct{324};
t1444 = ct{325};
t1445 = ct{326};
t1446 = ct{327};
t1448 = ct{328};
t1450 = ct{329};
t1451 = ct{330};
t1453 = ct{331};
t1455 = ct{332};
t1456 = ct{333};
t1457 = ct{334};
t1458 = ct{335};
t1459 = ct{336};
t1460 = ct{337};
t1461 = ct{338};
t1463 = ct{339};
t1465 = ct{340};
t1466 = ct{341};
t1467 = ct{342};
t1468 = ct{343};
t1469 = ct{344};
t1470 = ct{345};
t1473 = ct{346};
t1476 = ct{347};
t1477 = ct{348};
t1478 = ct{349};
t1479 = ct{350};
t1480 = ct{351};
t1481 = ct{352};
t1482 = ct{353};
t1483 = ct{354};
t1484 = ct{355};
t1486 = ct{356};
t1487 = ct{357};
t1488 = ct{358};
t1489 = ct{359};
t1491 = ct{360};
t1492 = ct{361};
t1493 = ct{362};
t1495 = ct{363};
t1496 = ct{364};
t1497 = ct{365};
t1498 = ct{366};
t15 = ct{367};
t1500 = ct{368};
t1505 = ct{369};
t1506 = ct{370};
t1508 = ct{371};
t1509 = ct{372};
t1510 = ct{373};
t1512 = ct{374};
t1513 = ct{375};
t1515 = ct{376};
t1516 = ct{377};
t1517 = ct{378};
t1518 = ct{379};
t1519 = ct{380};
t1520 = ct{381};
t1521 = ct{382};
t1522 = ct{383};
t1523 = ct{384};
t1525 = ct{385};
t1526 = ct{386};
t1527 = ct{387};
t1528 = ct{388};
t1529 = ct{389};
t1531 = ct{390};
t1532 = ct{391};
t1535 = ct{392};
t1537 = ct{393};
t1539 = ct{394};
t1540 = ct{395};
t1542 = ct{396};
t1543 = ct{397};
t1544 = ct{398};
t1546 = ct{399};
t1547 = ct{400};
t1548 = ct{401};
t1549 = ct{402};
t1550 = ct{403};
t1551 = ct{404};
t1552 = ct{405};
t1553 = ct{406};
t1555 = ct{407};
t1558 = ct{408};
t1559 = ct{409};
t1560 = ct{410};
t1561 = ct{411};
t1562 = ct{412};
t1563 = ct{413};
t1565 = ct{414};
t1566 = ct{415};
t1567 = ct{416};
t1568 = ct{417};
t1569 = ct{418};
t1570 = ct{419};
t1571 = ct{420};
t1574 = ct{421};
t1575 = ct{422};
t1576 = ct{423};
t1577 = ct{424};
t1578 = ct{425};
t1579 = ct{426};
t1580 = ct{427};
t1581 = ct{428};
t1582 = ct{429};
t1583 = ct{430};
t1584 = ct{431};
t1585 = ct{432};
t1586 = ct{433};
t1587 = ct{434};
t1589 = ct{435};
t1590 = ct{436};
t1591 = ct{437};
t1592 = ct{438};
t1593 = ct{439};
t1594 = ct{440};
t1595 = ct{441};
t1596 = ct{442};
t1597 = ct{443};
t1598 = ct{444};
t1599 = ct{445};
t160 = ct{446};
t1601 = ct{447};
t1602 = ct{448};
t1604 = ct{449};
t1605 = ct{450};
t1606 = ct{451};
t1609 = ct{452};
t161 = ct{453};
t1610 = ct{454};
t1612 = ct{455};
t1614 = ct{456};
t1615 = ct{457};
t1616 = ct{458};
t1617 = ct{459};
t1618 = ct{460};
t1619 = ct{461};
t162 = ct{462};
t1620 = ct{463};
t1621 = ct{464};
t1622 = ct{465};
t1623 = ct{466};
t1624 = ct{467};
t1625 = ct{468};
t1626 = ct{469};
t1627 = ct{470};
t1628 = ct{471};
t1630 = ct{472};
t1631 = ct{473};
t1632 = ct{474};
t1633 = ct{475};
t1634 = ct{476};
t1635 = ct{477};
t1636 = ct{478};
t1637 = ct{479};
t1638 = ct{480};
t1639 = ct{481};
t1640 = ct{482};
t1641 = ct{483};
t1642 = ct{484};
t1643 = ct{485};
t1644 = ct{486};
t1645 = ct{487};
t1646 = ct{488};
t1649 = ct{489};
t1651 = ct{490};
t1652 = ct{491};
t1653 = ct{492};
t1654 = ct{493};
t1655 = ct{494};
t1656 = ct{495};
t1657 = ct{496};
t1658 = ct{497};
t1659 = ct{498};
t1660 = ct{499};
t1661 = ct{500};
t1662 = ct{501};
t1663 = ct{502};
t1664 = ct{503};
t1665 = ct{504};
t1666 = ct{505};
t1667 = ct{506};
t1668 = ct{507};
t1669 = ct{508};
t1671 = ct{509};
t1672 = ct{510};
t1674 = ct{511};
t1675 = ct{512};
t1676 = ct{513};
t1677 = ct{514};
t1678 = ct{515};
t1679 = ct{516};
t1680 = ct{517};
t1681 = ct{518};
t1682 = ct{519};
t1683 = ct{520};
t1684 = ct{521};
t1685 = ct{522};
t1686 = ct{523};
t1687 = ct{524};
t1688 = ct{525};
t1689 = ct{526};
t1690 = ct{527};
t1691 = ct{528};
t1692 = ct{529};
t1693 = ct{530};
t1694 = ct{531};
t1695 = ct{532};
t1696 = ct{533};
t1697 = ct{534};
t1698 = ct{535};
t1699 = ct{536};
t1700 = ct{537};
t1701 = ct{538};
t1702 = ct{539};
t1703 = ct{540};
t1704 = ct{541};
t1705 = ct{542};
t1706 = ct{543};
t1711 = ct{544};
t1715 = ct{545};
t1716 = ct{546};
t1718 = ct{547};
t1719 = ct{548};
t1720 = ct{549};
t1721 = ct{550};
t1722 = ct{551};
t1723 = ct{552};
t1725 = ct{553};
t1726 = ct{554};
t1727 = ct{555};
t1729 = ct{556};
t1730 = ct{557};
t1731 = ct{558};
t1732 = ct{559};
t1733 = ct{560};
t1734 = ct{561};
t1735 = ct{562};
t1736 = ct{563};
t1737 = ct{564};
t1739 = ct{565};
t1740 = ct{566};
t1741 = ct{567};
t1742 = ct{568};
t1743 = ct{569};
t1744 = ct{570};
t1745 = ct{571};
t1746 = ct{572};
t1747 = ct{573};
t1748 = ct{574};
t1749 = ct{575};
t1750 = ct{576};
t1751 = ct{577};
t1753 = ct{578};
t1755 = ct{579};
t1756 = ct{580};
t1758 = ct{581};
t1759 = ct{582};
t1761 = ct{583};
t1762 = ct{584};
t1763 = ct{585};
t1764 = ct{586};
t1765 = ct{587};
t1769 = ct{588};
t1770 = ct{589};
t1771 = ct{590};
t1774 = ct{591};
t1777 = ct{592};
t1778 = ct{593};
t1779 = ct{594};
t1780 = ct{595};
t1781 = ct{596};
t1783 = ct{597};
t1784 = ct{598};
t1785 = ct{599};
t1786 = ct{600};
t1787 = ct{601};
t1788 = ct{602};
t1789 = ct{603};
t1790 = ct{604};
t1791 = ct{605};
t1792 = ct{606};
t1796 = ct{607};
t1798 = ct{608};
t1799 = ct{609};
t1800 = ct{610};
t1801 = ct{611};
t1802 = ct{612};
t1803 = ct{613};
t1806 = ct{614};
t1809 = ct{615};
t1810 = ct{616};
t1811 = ct{617};
t1812 = ct{618};
t1813 = ct{619};
t1814 = ct{620};
t1815 = ct{621};
t1816 = ct{622};
t1817 = ct{623};
t1819 = ct{624};
t1820 = ct{625};
t1821 = ct{626};
t1822 = ct{627};
t1823 = ct{628};
t1824 = ct{629};
t1825 = ct{630};
t1826 = ct{631};
t1827 = ct{632};
t1828 = ct{633};
t1829 = ct{634};
t1830 = ct{635};
t1831 = ct{636};
t1832 = ct{637};
t1833 = ct{638};
t1834 = ct{639};
t1835 = ct{640};
t1836 = ct{641};
t1839 = ct{642};
t1841 = ct{643};
t1842 = ct{644};
t1843 = ct{645};
t1844 = ct{646};
t1845 = ct{647};
t1846 = ct{648};
t1847 = ct{649};
t1848 = ct{650};
t1849 = ct{651};
t1851 = ct{652};
t1852 = ct{653};
t1855 = ct{654};
t1856 = ct{655};
t1857 = ct{656};
t1858 = ct{657};
t1859 = ct{658};
t1860 = ct{659};
t1862 = ct{660};
t1863 = ct{661};
t1864 = ct{662};
t1865 = ct{663};
t1866 = ct{664};
t1867 = ct{665};
t1870 = ct{666};
t1871 = ct{667};
t1872 = ct{668};
t1873 = ct{669};
t1874 = ct{670};
t1875 = ct{671};
t1877 = ct{672};
t1878 = ct{673};
t1880 = ct{674};
t1881 = ct{675};
t1882 = ct{676};
t1883 = ct{677};
t1884 = ct{678};
t1885 = ct{679};
t1887 = ct{680};
t1888 = ct{681};
t1890 = ct{682};
t1891 = ct{683};
t1893 = ct{684};
t1894 = ct{685};
t1895 = ct{686};
t1896 = ct{687};
t1898 = ct{688};
t1899 = ct{689};
t1900 = ct{690};
t1902 = ct{691};
t1904 = ct{692};
t1905 = ct{693};
t1906 = ct{694};
t1907 = ct{695};
t1908 = ct{696};
t1909 = ct{697};
t1910 = ct{698};
t1911 = ct{699};
t1912 = ct{700};
t1913 = ct{701};
t1914 = ct{702};
t1915 = ct{703};
t1916 = ct{704};
t1917 = ct{705};
t1918 = ct{706};
t1919 = ct{707};
t1920 = ct{708};
t1921 = ct{709};
t1922 = ct{710};
t1923 = ct{711};
t1924 = ct{712};
t1926 = ct{713};
t1928 = ct{714};
t1929 = ct{715};
t1930 = ct{716};
t1931 = ct{717};
t1932 = ct{718};
t1933 = ct{719};
t1934 = ct{720};
t1935 = ct{721};
t1937 = ct{722};
t1938 = ct{723};
t1939 = ct{724};
t1940 = ct{725};
t1941 = ct{726};
t1942 = ct{727};
t1943 = ct{728};
t1945 = ct{729};
t1946 = ct{730};
t1947 = ct{731};
t1948 = ct{732};
t1949 = ct{733};
t195 = ct{734};
t1950 = ct{735};
t1951 = ct{736};
t1952 = ct{737};
t1953 = ct{738};
t1955 = ct{739};
t1956 = ct{740};
t1957 = ct{741};
t1959 = ct{742};
t1960 = ct{743};
t1961 = ct{744};
t1962 = ct{745};
t1963 = ct{746};
t1964 = ct{747};
t1965 = ct{748};
t1966 = ct{749};
t1967 = ct{750};
t1968 = ct{751};
t1969 = ct{752};
t197 = ct{753};
t1970 = ct{754};
t1971 = ct{755};
t1973 = ct{756};
t1974 = ct{757};
t1975 = ct{758};
t1976 = ct{759};
t1977 = ct{760};
t1978 = ct{761};
t1979 = ct{762};
t1980 = ct{763};
t1981 = ct{764};
t1982 = ct{765};
t1983 = ct{766};
t1984 = ct{767};
t1985 = ct{768};
t1986 = ct{769};
t1987 = ct{770};
t1988 = ct{771};
t1989 = ct{772};
t1990 = ct{773};
t1991 = ct{774};
t1992 = ct{775};
t1993 = ct{776};
t1994 = ct{777};
t1995 = ct{778};
t1998 = ct{779};
t1999 = ct{780};
t2 = ct{781};
t2000 = ct{782};
t2001 = ct{783};
t2002 = ct{784};
t2004 = ct{785};
t2005 = ct{786};
t2006 = ct{787};
t2007 = ct{788};
t2008 = ct{789};
t2009 = ct{790};
t2010 = ct{791};
t2011 = ct{792};
t2012 = ct{793};
t2014 = ct{794};
t2015 = ct{795};
t2016 = ct{796};
t2017 = ct{797};
t2018 = ct{798};
t2019 = ct{799};
t2020 = ct{800};
t2023 = ct{801};
t2024 = ct{802};
t2025 = ct{803};
t2026 = ct{804};
t2028 = ct{805};
t2030 = ct{806};
t2032 = ct{807};
t2033 = ct{808};
t2035 = ct{809};
t2037 = ct{810};
t2039 = ct{811};
t2041 = ct{812};
t2042 = ct{813};
t2043 = ct{814};
t2045 = ct{815};
t2046 = ct{816};
t2047 = ct{817};
t2048 = ct{818};
t2049 = ct{819};
t2050 = ct{820};
t2053 = ct{821};
t2057 = ct{822};
t2058 = ct{823};
t2059 = ct{824};
t2060 = ct{825};
t2061 = ct{826};
t2062 = ct{827};
t2063 = ct{828};
t2064 = ct{829};
t2065 = ct{830};
t2066 = ct{831};
t2067 = ct{832};
t2068 = ct{833};
t2069 = ct{834};
t2070 = ct{835};
t2072 = ct{836};
t2073 = ct{837};
t2074 = ct{838};
t2075 = ct{839};
t2076 = ct{840};
t2078 = ct{841};
t2079 = ct{842};
t2080 = ct{843};
t2081 = ct{844};
t2082 = ct{845};
t2083 = ct{846};
t2084 = ct{847};
t2085 = ct{848};
t2087 = ct{849};
t2088 = ct{850};
t2090 = ct{851};
t2091 = ct{852};
t2092 = ct{853};
t2093 = ct{854};
t2094 = ct{855};
t2095 = ct{856};
t2096 = ct{857};
t2097 = ct{858};
t2098 = ct{859};
t2099 = ct{860};
t2100 = ct{861};
t2101 = ct{862};
t2102 = ct{863};
t2103 = ct{864};
t2104 = ct{865};
t2105 = ct{866};
t2106 = ct{867};
t2108 = ct{868};
t2109 = ct{869};
t2110 = ct{870};
t2111 = ct{871};
t2112 = ct{872};
t2113 = ct{873};
t2114 = ct{874};
t2115 = ct{875};
t2116 = ct{876};
t2117 = ct{877};
t2118 = ct{878};
t2119 = ct{879};
t2120 = ct{880};
t2121 = ct{881};
t2122 = ct{882};
t2123 = ct{883};
t2124 = ct{884};
t2125 = ct{885};
t2126 = ct{886};
t2127 = ct{887};
t2129 = ct{888};
t2130 = ct{889};
t2131 = ct{890};
t2132 = ct{891};
t2133 = ct{892};
t2134 = ct{893};
t2135 = ct{894};
t2136 = ct{895};
t2137 = ct{896};
t214 = ct{897};
t2141 = ct{898};
t2142 = ct{899};
t2143 = ct{900};
t2144 = ct{901};
t2147 = ct{902};
t2148 = ct{903};
t2149 = ct{904};
t2150 = ct{905};
t2151 = ct{906};
t2152 = ct{907};
t2153 = ct{908};
t2154 = ct{909};
t2155 = ct{910};
t2156 = ct{911};
t2157 = ct{912};
t2158 = ct{913};
t2160 = ct{914};
t2161 = ct{915};
t2164 = ct{916};
t2165 = ct{917};
t2166 = ct{918};
t2167 = ct{919};
t2169 = ct{920};
t2170 = ct{921};
t2171 = ct{922};
t2172 = ct{923};
t2174 = ct{924};
t2175 = ct{925};
t2176 = ct{926};
t2177 = ct{927};
t2178 = ct{928};
t2179 = ct{929};
t2181 = ct{930};
t2182 = ct{931};
t2183 = ct{932};
t2186 = ct{933};
t2187 = ct{934};
t2188 = ct{935};
t2189 = ct{936};
t2190 = ct{937};
t2191 = ct{938};
t2192 = ct{939};
t2193 = ct{940};
t2194 = ct{941};
t2196 = ct{942};
t2197 = ct{943};
t2199 = ct{944};
t2200 = ct{945};
t2201 = ct{946};
t2202 = ct{947};
t2203 = ct{948};
t2204 = ct{949};
t2205 = ct{950};
t2206 = ct{951};
t2208 = ct{952};
t2209 = ct{953};
t2210 = ct{954};
t2211 = ct{955};
t2212 = ct{956};
t2213 = ct{957};
t2214 = ct{958};
t2215 = ct{959};
t2216 = ct{960};
t2217 = ct{961};
t2218 = ct{962};
t2219 = ct{963};
t2220 = ct{964};
t2221 = ct{965};
t2222 = ct{966};
t2223 = ct{967};
t2224 = ct{968};
t2225 = ct{969};
t2227 = ct{970};
t2228 = ct{971};
t2229 = ct{972};
t2230 = ct{973};
t2232 = ct{974};
t2233 = ct{975};
t2235 = ct{976};
t2236 = ct{977};
t2237 = ct{978};
t2238 = ct{979};
t2239 = ct{980};
t2240 = ct{981};
t2241 = ct{982};
t2242 = ct{983};
t2245 = ct{984};
t2246 = ct{985};
t2247 = ct{986};
t2248 = ct{987};
t2249 = ct{988};
t2251 = ct{989};
t2252 = ct{990};
t2253 = ct{991};
t2254 = ct{992};
t2255 = ct{993};
t2257 = ct{994};
t2258 = ct{995};
t2259 = ct{996};
t2260 = ct{997};
t2262 = ct{998};
t2263 = ct{999};
t2265 = ct{1000};
t2267 = ct{1001};
t2268 = ct{1002};
t2269 = ct{1003};
t2270 = ct{1004};
t2271 = ct{1005};
t2272 = ct{1006};
t2274 = ct{1007};
t2276 = ct{1008};
t2277 = ct{1009};
t2281 = ct{1010};
t2284 = ct{1011};
t2285 = ct{1012};
t2286 = ct{1013};
t2287 = ct{1014};
t2288 = ct{1015};
t2289 = ct{1016};
t2290 = ct{1017};
t2292 = ct{1018};
t2293 = ct{1019};
t2294 = ct{1020};
t2296 = ct{1021};
t2298 = ct{1022};
t2299 = ct{1023};
t2300 = ct{1024};
t2303 = ct{1025};
t2304 = ct{1026};
t2305 = ct{1027};
t2307 = ct{1028};
t2308 = ct{1029};
t2309 = ct{1030};
t2312 = ct{1031};
t2313 = ct{1032};
t2314 = ct{1033};
t2316 = ct{1034};
t2317 = ct{1035};
t2318 = ct{1036};
t2319 = ct{1037};
t2320 = ct{1038};
t2321 = ct{1039};
t2322 = ct{1040};
t2323 = ct{1041};
t2324 = ct{1042};
t2325 = ct{1043};
t2327 = ct{1044};
t2328 = ct{1045};
t2329 = ct{1046};
t2330 = ct{1047};
t2331 = ct{1048};
t2333 = ct{1049};
t2334 = ct{1050};
t2335 = ct{1051};
t2336 = ct{1052};
t2338 = ct{1053};
t2339 = ct{1054};
t2340 = ct{1055};
t2341 = ct{1056};
t2342 = ct{1057};
t2343 = ct{1058};
t2344 = ct{1059};
t2345 = ct{1060};
t2346 = ct{1061};
t2347 = ct{1062};
t2348 = ct{1063};
t2349 = ct{1064};
t2350 = ct{1065};
t2351 = ct{1066};
t2352 = ct{1067};
t2354 = ct{1068};
t2355 = ct{1069};
t2356 = ct{1070};
t2358 = ct{1071};
t2360 = ct{1072};
t2361 = ct{1073};
t2362 = ct{1074};
t2363 = ct{1075};
t2364 = ct{1076};
t2365 = ct{1077};
t2368 = ct{1078};
t2369 = ct{1079};
t2370 = ct{1080};
t2371 = ct{1081};
t2373 = ct{1082};
t2374 = ct{1083};
t2375 = ct{1084};
t2376 = ct{1085};
t2377 = ct{1086};
t2378 = ct{1087};
t2380 = ct{1088};
t2381 = ct{1089};
t2382 = ct{1090};
t2385 = ct{1091};
t2386 = ct{1092};
t2387 = ct{1093};
t2388 = ct{1094};
t2389 = ct{1095};
t2390 = ct{1096};
t2392 = ct{1097};
t2396 = ct{1098};
t2397 = ct{1099};
t2399 = ct{1100};
t24 = ct{1101};
t2400 = ct{1102};
t2401 = ct{1103};
t2403 = ct{1104};
t2404 = ct{1105};
t2406 = ct{1106};
t2407 = ct{1107};
t2408 = ct{1108};
t2409 = ct{1109};
t2410 = ct{1110};
t2411 = ct{1111};
t2412 = ct{1112};
t2413 = ct{1113};
t2414 = ct{1114};
t2417 = ct{1115};
t2419 = ct{1116};
t2420 = ct{1117};
t2422 = ct{1118};
t2423 = ct{1119};
t2425 = ct{1120};
t2426 = ct{1121};
t2427 = ct{1122};
t2428 = ct{1123};
t2429 = ct{1124};
t2430 = ct{1125};
t2431 = ct{1126};
t2432 = ct{1127};
t2433 = ct{1128};
t2434 = ct{1129};
t2435 = ct{1130};
t2436 = ct{1131};
t2437 = ct{1132};
t2438 = ct{1133};
t2439 = ct{1134};
t2442 = ct{1135};
t2443 = ct{1136};
t2444 = ct{1137};
t2445 = ct{1138};
t2446 = ct{1139};
t2447 = ct{1140};
t2448 = ct{1141};
t2449 = ct{1142};
t2452 = ct{1143};
t2453 = ct{1144};
t2454 = ct{1145};
t2455 = ct{1146};
t2457 = ct{1147};
t2458 = ct{1148};
t2459 = ct{1149};
t2460 = ct{1150};
t2461 = ct{1151};
t2462 = ct{1152};
t2463 = ct{1153};
t2464 = ct{1154};
t2465 = ct{1155};
t2466 = ct{1156};
t2467 = ct{1157};
t2468 = ct{1158};
t2469 = ct{1159};
t2470 = ct{1160};
t2471 = ct{1161};
t2472 = ct{1162};
t2474 = ct{1163};
t2476 = ct{1164};
t2479 = ct{1165};
t2480 = ct{1166};
t2483 = ct{1167};
t2484 = ct{1168};
t2485 = ct{1169};
t2486 = ct{1170};
t2487 = ct{1171};
t2488 = ct{1172};
t2489 = ct{1173};
t2492 = ct{1174};
t2495 = ct{1175};
t2496 = ct{1176};
t2498 = ct{1177};
t25 = ct{1178};
t2502 = ct{1179};
t2503 = ct{1180};
t2504 = ct{1181};
t2505 = ct{1182};
t2506 = ct{1183};
t2508 = ct{1184};
t2509 = ct{1185};
t2511 = ct{1186};
t2512 = ct{1187};
t2513 = ct{1188};
t2514 = ct{1189};
t2515 = ct{1190};
t2516 = ct{1191};
t2518 = ct{1192};
t2519 = ct{1193};
t2520 = ct{1194};
t2521 = ct{1195};
t2522 = ct{1196};
t2523 = ct{1197};
t2524 = ct{1198};
t2525 = ct{1199};
t2526 = ct{1200};
t2527 = ct{1201};
t2528 = ct{1202};
t2529 = ct{1203};
t2530 = ct{1204};
t2531 = ct{1205};
t2532 = ct{1206};
t2533 = ct{1207};
t2534 = ct{1208};
t2535 = ct{1209};
t2536 = ct{1210};
t2537 = ct{1211};
t2538 = ct{1212};
t2539 = ct{1213};
t2541 = ct{1214};
t2542 = ct{1215};
t2543 = ct{1216};
t2544 = ct{1217};
t2545 = ct{1218};
t2546 = ct{1219};
t2547 = ct{1220};
t2548 = ct{1221};
t2549 = ct{1222};
t2550 = ct{1223};
t2551 = ct{1224};
t2552 = ct{1225};
t2555 = ct{1226};
t2556 = ct{1227};
t2559 = ct{1228};
t2560 = ct{1229};
t2561 = ct{1230};
t2562 = ct{1231};
t2563 = ct{1232};
t2564 = ct{1233};
t2565 = ct{1234};
t2566 = ct{1235};
t2567 = ct{1236};
t2568 = ct{1237};
t2569 = ct{1238};
t2570 = ct{1239};
t2571 = ct{1240};
t2573 = ct{1241};
t2574 = ct{1242};
t2575 = ct{1243};
t2576 = ct{1244};
t2577 = ct{1245};
t2578 = ct{1246};
t2579 = ct{1247};
t2581 = ct{1248};
t2582 = ct{1249};
t2583 = ct{1250};
t2584 = ct{1251};
t2585 = ct{1252};
t2587 = ct{1253};
t2588 = ct{1254};
t2589 = ct{1255};
t259 = ct{1256};
t2590 = ct{1257};
t2591 = ct{1258};
t2593 = ct{1259};
t2594 = ct{1260};
t2595 = ct{1261};
t2596 = ct{1262};
t2597 = ct{1263};
t2598 = ct{1264};
t2599 = ct{1265};
t26 = ct{1266};
t260 = ct{1267};
t2600 = ct{1268};
t2602 = ct{1269};
t2605 = ct{1270};
t2606 = ct{1271};
t2607 = ct{1272};
t2610 = ct{1273};
t2611 = ct{1274};
t2612 = ct{1275};
t2613 = ct{1276};
t2615 = ct{1277};
t2616 = ct{1278};
t2617 = ct{1279};
t2619 = ct{1280};
t2620 = ct{1281};
t2621 = ct{1282};
t2623 = ct{1283};
t2624 = ct{1284};
t2627 = ct{1285};
t2629 = ct{1286};
t2630 = ct{1287};
t2631 = ct{1288};
t2632 = ct{1289};
t2634 = ct{1290};
t2635 = ct{1291};
t2636 = ct{1292};
t2637 = ct{1293};
t2638 = ct{1294};
t2640 = ct{1295};
t2641 = ct{1296};
t2642 = ct{1297};
t2643 = ct{1298};
t2644 = ct{1299};
t2645 = ct{1300};
t2646 = ct{1301};
t2647 = ct{1302};
t2648 = ct{1303};
t2649 = ct{1304};
t2650 = ct{1305};
t2654 = ct{1306};
t2656 = ct{1307};
t2657 = ct{1308};
t2658 = ct{1309};
t2660 = ct{1310};
t2661 = ct{1311};
t2662 = ct{1312};
t2663 = ct{1313};
t2665 = ct{1314};
t2666 = ct{1315};
t2667 = ct{1316};
t2668 = ct{1317};
t2669 = ct{1318};
t2671 = ct{1319};
t2672 = ct{1320};
t2673 = ct{1321};
t2674 = ct{1322};
t2675 = ct{1323};
t2677 = ct{1324};
t2678 = ct{1325};
t2679 = ct{1326};
t2681 = ct{1327};
t2682 = ct{1328};
t2684 = ct{1329};
t2685 = ct{1330};
t2688 = ct{1331};
t2689 = ct{1332};
t2691 = ct{1333};
t2692 = ct{1334};
t2695 = ct{1335};
t2696 = ct{1336};
t2698 = ct{1337};
t2699 = ct{1338};
t27 = ct{1339};
t2700 = ct{1340};
t2704 = ct{1341};
t2705 = ct{1342};
t2706 = ct{1343};
t2707 = ct{1344};
t2708 = ct{1345};
t2710 = ct{1346};
t2711 = ct{1347};
t2712 = ct{1348};
t2714 = ct{1349};
t2715 = ct{1350};
t2717 = ct{1351};
t2718 = ct{1352};
t2722 = ct{1353};
t2723 = ct{1354};
t2725 = ct{1355};
t2726 = ct{1356};
t2727 = ct{1357};
t2728 = ct{1358};
t2730 = ct{1359};
t2731 = ct{1360};
t2732 = ct{1361};
t2733 = ct{1362};
t2735 = ct{1363};
t2736 = ct{1364};
t2737 = ct{1365};
t2738 = ct{1366};
t2739 = ct{1367};
t2740 = ct{1368};
t2742 = ct{1369};
t2743 = ct{1370};
t2744 = ct{1371};
t2746 = ct{1372};
t2747 = ct{1373};
t2748 = ct{1374};
t2749 = ct{1375};
t2750 = ct{1376};
t2751 = ct{1377};
t2752 = ct{1378};
t2754 = ct{1379};
t2755 = ct{1380};
t2756 = ct{1381};
t2758 = ct{1382};
t2759 = ct{1383};
t276 = ct{1384};
t2760 = ct{1385};
t2761 = ct{1386};
t2763 = ct{1387};
t2764 = ct{1388};
t2765 = ct{1389};
t2766 = ct{1390};
t2768 = ct{1391};
t2769 = ct{1392};
t277 = ct{1393};
t2770 = ct{1394};
t2771 = ct{1395};
t2772 = ct{1396};
t2774 = ct{1397};
t2775 = ct{1398};
t2776 = ct{1399};
t2778 = ct{1400};
t2779 = ct{1401};
t2781 = ct{1402};
t2782 = ct{1403};
t2783 = ct{1404};
t2785 = ct{1405};
t2786 = ct{1406};
t2787 = ct{1407};
t2788 = ct{1408};
t2790 = ct{1409};
t2791 = ct{1410};
t2792 = ct{1411};
t2793 = ct{1412};
t2795 = ct{1413};
t2796 = ct{1414};
t2797 = ct{1415};
t2798 = ct{1416};
t2799 = ct{1417};
t28 = ct{1418};
t2800 = ct{1419};
t2802 = ct{1420};
t2803 = ct{1421};
t2804 = ct{1422};
t2806 = ct{1423};
t2807 = ct{1424};
t2811 = ct{1425};
t2813 = ct{1426};
t2814 = ct{1427};
t2816 = ct{1428};
t2817 = ct{1429};
t2818 = ct{1430};
t2819 = ct{1431};
t2821 = ct{1432};
t2823 = ct{1433};
t2824 = ct{1434};
t2825 = ct{1435};
t2826 = ct{1436};
t2827 = ct{1437};
t2828 = ct{1438};
t2829 = ct{1439};
t283 = ct{1440};
t2830 = ct{1441};
t2831 = ct{1442};
t2832 = ct{1443};
t2833 = ct{1444};
t2834 = ct{1445};
t2835 = ct{1446};
t2836 = ct{1447};
t2837 = ct{1448};
t2838 = ct{1449};
t2839 = ct{1450};
t284 = ct{1451};
t2841 = ct{1452};
t2842 = ct{1453};
t2843 = ct{1454};
t2844 = ct{1455};
t2845 = ct{1456};
t2846 = ct{1457};
t2847 = ct{1458};
t2848 = ct{1459};
t2849 = ct{1460};
t285 = ct{1461};
t2851 = ct{1462};
t2852 = ct{1463};
t2853 = ct{1464};
t2857 = ct{1465};
t2858 = ct{1466};
t2859 = ct{1467};
t286 = ct{1468};
t2860 = ct{1469};
t2861 = ct{1470};
t2862 = ct{1471};
t2864 = ct{1472};
t2865 = ct{1473};
t2866 = ct{1474};
t2867 = ct{1475};
t2868 = ct{1476};
t2869 = ct{1477};
t287 = ct{1478};
t2870 = ct{1479};
t2871 = ct{1480};
t2872 = ct{1481};
t2874 = ct{1482};
t2875 = ct{1483};
t2876 = ct{1484};
t2877 = ct{1485};
t2878 = ct{1486};
t2879 = ct{1487};
t288 = ct{1488};
t2880 = ct{1489};
t2881 = ct{1490};
t2882 = ct{1491};
t2883 = ct{1492};
t2884 = ct{1493};
t2885 = ct{1494};
t2886 = ct{1495};
t2887 = ct{1496};
t2889 = ct{1497};
t289 = ct{1498};
t2890 = ct{1499};
t2892 = ct{1500};
t2893 = ct{1501};
t2895 = ct{1502};
t2896 = ct{1503};
t2897 = ct{1504};
t2898 = ct{1505};
t2899 = ct{1506};
t290 = ct{1507};
t2900 = ct{1508};
t2901 = ct{1509};
t2902 = ct{1510};
t2903 = ct{1511};
t2904 = ct{1512};
t2906 = ct{1513};
t2907 = ct{1514};
t2909 = ct{1515};
t291 = ct{1516};
t2912 = ct{1517};
t2913 = ct{1518};
t2914 = ct{1519};
t2915 = ct{1520};
t2916 = ct{1521};
t2917 = ct{1522};
t2918 = ct{1523};
t2919 = ct{1524};
t292 = ct{1525};
t2920 = ct{1526};
t2921 = ct{1527};
t2922 = ct{1528};
t2923 = ct{1529};
t2924 = ct{1530};
t2925 = ct{1531};
t2926 = ct{1532};
t2927 = ct{1533};
t2928 = ct{1534};
t2929 = ct{1535};
t293 = ct{1536};
t2932 = ct{1537};
t2933 = ct{1538};
t2934 = ct{1539};
t2935 = ct{1540};
t2936 = ct{1541};
t2937 = ct{1542};
t2938 = ct{1543};
t294 = ct{1544};
t2940 = ct{1545};
t2941 = ct{1546};
t2942 = ct{1547};
t2943 = ct{1548};
t2944 = ct{1549};
t2945 = ct{1550};
t2946 = ct{1551};
t2947 = ct{1552};
t2949 = ct{1553};
t2950 = ct{1554};
t2951 = ct{1555};
t2952 = ct{1556};
t2954 = ct{1557};
t2955 = ct{1558};
t2956 = ct{1559};
t2957 = ct{1560};
t2959 = ct{1561};
t2960 = ct{1562};
t2961 = ct{1563};
t2962 = ct{1564};
t2963 = ct{1565};
t2964 = ct{1566};
t2966 = ct{1567};
t2967 = ct{1568};
t2969 = ct{1569};
t2972 = ct{1570};
t2975 = ct{1571};
t2976 = ct{1572};
t2977 = ct{1573};
t2978 = ct{1574};
t2979 = ct{1575};
t2981 = ct{1576};
t2982 = ct{1577};
t2985 = ct{1578};
t2986 = ct{1579};
t2987 = ct{1580};
t2988 = ct{1581};
t2989 = ct{1582};
t2992 = ct{1583};
t2994 = ct{1584};
t2995 = ct{1585};
t2996 = ct{1586};
t2997 = ct{1587};
t2998 = ct{1588};
t2999 = ct{1589};
t3 = ct{1590};
t30 = ct{1591};
t3003 = ct{1592};
t3004 = ct{1593};
t3006 = ct{1594};
t3007 = ct{1595};
t3008 = ct{1596};
t3009 = ct{1597};
t3010 = ct{1598};
t3011 = ct{1599};
t3012 = ct{1600};
t3016 = ct{1601};
t3017 = ct{1602};
t3019 = ct{1603};
t3020 = ct{1604};
t3022 = ct{1605};
t3023 = ct{1606};
t3027 = ct{1607};
t3030 = ct{1608};
t3031 = ct{1609};
t3032 = ct{1610};
t3033 = ct{1611};
t3034 = ct{1612};
t3035 = ct{1613};
t3036 = ct{1614};
t3037 = ct{1615};
t3038 = ct{1616};
t3039 = ct{1617};
t304 = ct{1618};
t3041 = ct{1619};
t3042 = ct{1620};
t3043 = ct{1621};
t3044 = ct{1622};
t3045 = ct{1623};
t3046 = ct{1624};
t3047 = ct{1625};
t3049 = ct{1626};
t3050 = ct{1627};
t3051 = ct{1628};
t3054 = ct{1629};
t3059 = ct{1630};
t3060 = ct{1631};
t3061 = ct{1632};
t3062 = ct{1633};
t3063 = ct{1634};
t3064 = ct{1635};
t3065 = ct{1636};
t3066 = ct{1637};
t3069 = ct{1638};
t3070 = ct{1639};
t3071 = ct{1640};
t3072 = ct{1641};
t3073 = ct{1642};
t3074 = ct{1643};
t3075 = ct{1644};
t3076 = ct{1645};
t3077 = ct{1646};
t3078 = ct{1647};
t3080 = ct{1648};
t3081 = ct{1649};
t3082 = ct{1650};
t3083 = ct{1651};
t3084 = ct{1652};
t3085 = ct{1653};
t3087 = ct{1654};
t3089 = ct{1655};
t3090 = ct{1656};
t3091 = ct{1657};
t3092 = ct{1658};
t3093 = ct{1659};
t3094 = ct{1660};
t3095 = ct{1661};
t3096 = ct{1662};
t3097 = ct{1663};
t3098 = ct{1664};
t3099 = ct{1665};
t3100 = ct{1666};
t3101 = ct{1667};
t3102 = ct{1668};
t3105 = ct{1669};
t3106 = ct{1670};
t3107 = ct{1671};
t3108 = ct{1672};
t3109 = ct{1673};
t3110 = ct{1674};
t3112 = ct{1675};
t3113 = ct{1676};
t3114 = ct{1677};
t3115 = ct{1678};
t3117 = ct{1679};
t3119 = ct{1680};
t3122 = ct{1681};
t3123 = ct{1682};
t3124 = ct{1683};
t3127 = ct{1684};
t3128 = ct{1685};
t3130 = ct{1686};
t3131 = ct{1687};
t3132 = ct{1688};
t3133 = ct{1689};
t3134 = ct{1690};
t3135 = ct{1691};
t3136 = ct{1692};
t3138 = ct{1693};
t3139 = ct{1694};
t3143 = ct{1695};
t3145 = ct{1696};
t3146 = ct{1697};
t3147 = ct{1698};
t3149 = ct{1699};
t3150 = ct{1700};
t3151 = ct{1701};
t3153 = ct{1702};
t3156 = ct{1703};
t3157 = ct{1704};
t3158 = ct{1705};
t3160 = ct{1706};
t3162 = ct{1707};
t3163 = ct{1708};
t3164 = ct{1709};
t3165 = ct{1710};
t3166 = ct{1711};
t3167 = ct{1712};
t3169 = ct{1713};
t3170 = ct{1714};
t3171 = ct{1715};
t3173 = ct{1716};
t3174 = ct{1717};
t3175 = ct{1718};
t3176 = ct{1719};
t3177 = ct{1720};
t3178 = ct{1721};
t3179 = ct{1722};
t3180 = ct{1723};
t3181 = ct{1724};
t3184 = ct{1725};
t3185 = ct{1726};
t3186 = ct{1727};
t3187 = ct{1728};
t3189 = ct{1729};
t3192 = ct{1730};
t3195 = ct{1731};
t3196 = ct{1732};
t3197 = ct{1733};
t3198 = ct{1734};
t3199 = ct{1735};
t3200 = ct{1736};
t3203 = ct{1737};
t3204 = ct{1738};
t3206 = ct{1739};
t3207 = ct{1740};
t3210 = ct{1741};
t3211 = ct{1742};
t3212 = ct{1743};
t3213 = ct{1744};
t3214 = ct{1745};
t3215 = ct{1746};
t3216 = ct{1747};
t3217 = ct{1748};
t3218 = ct{1749};
t3220 = ct{1750};
t3221 = ct{1751};
t3222 = ct{1752};
t3223 = ct{1753};
t3224 = ct{1754};
t3225 = ct{1755};
t3226 = ct{1756};
t3228 = ct{1757};
t3229 = ct{1758};
t3230 = ct{1759};
t3233 = ct{1760};
t3235 = ct{1761};
t3236 = ct{1762};
t3238 = ct{1763};
t3239 = ct{1764};
t3240 = ct{1765};
t3241 = ct{1766};
t3243 = ct{1767};
t3244 = ct{1768};
t3245 = ct{1769};
t3246 = ct{1770};
t3247 = ct{1771};
t3248 = ct{1772};
t3250 = ct{1773};
t3252 = ct{1774};
t3253 = ct{1775};
t3255 = ct{1776};
t3256 = ct{1777};
t3260 = ct{1778};
t3261 = ct{1779};
t3263 = ct{1780};
t3265 = ct{1781};
t3266 = ct{1782};
t3270 = ct{1783};
t3271 = ct{1784};
t3272 = ct{1785};
t3273 = ct{1786};
t3274 = ct{1787};
t3275 = ct{1788};
t3276 = ct{1789};
t3277 = ct{1790};
t3278 = ct{1791};
t3279 = ct{1792};
t3280 = ct{1793};
t3281 = ct{1794};
t3282 = ct{1795};
t3283 = ct{1796};
t3284 = ct{1797};
t3285 = ct{1798};
t3286 = ct{1799};
t3287 = ct{1800};
t3288 = ct{1801};
t3289 = ct{1802};
t3290 = ct{1803};
t3291 = ct{1804};
t3294 = ct{1805};
t3295 = ct{1806};
t3296 = ct{1807};
t33 = ct{1808};
t3300 = ct{1809};
t3301 = ct{1810};
t3303 = ct{1811};
t3304 = ct{1812};
t3305 = ct{1813};
t3306 = ct{1814};
t3307 = ct{1815};
t3311 = ct{1816};
t3312 = ct{1817};
t3315 = ct{1818};
t3317 = ct{1819};
t3319 = ct{1820};
t3320 = ct{1821};
t3321 = ct{1822};
t3322 = ct{1823};
t3323 = ct{1824};
t3325 = ct{1825};
t3326 = ct{1826};
t3330 = ct{1827};
t3331 = ct{1828};
t3332 = ct{1829};
t3333 = ct{1830};
t3334 = ct{1831};
t3337 = ct{1832};
t3338 = ct{1833};
t3339 = ct{1834};
t3340 = ct{1835};
t3341 = ct{1836};
t3346 = ct{1837};
t3348 = ct{1838};
t3350 = ct{1839};
t3351 = ct{1840};
t3353 = ct{1841};
t3354 = ct{1842};
t3356 = ct{1843};
t3357 = ct{1844};
t3358 = ct{1845};
t3359 = ct{1846};
t3360 = ct{1847};
t3361 = ct{1848};
t3363 = ct{1849};
t3364 = ct{1850};
t3365 = ct{1851};
t3366 = ct{1852};
t3367 = ct{1853};
t3368 = ct{1854};
t3369 = ct{1855};
t3370 = ct{1856};
t3371 = ct{1857};
t3372 = ct{1858};
t3373 = ct{1859};
t3374 = ct{1860};
t3375 = ct{1861};
t3376 = ct{1862};
t3378 = ct{1863};
t3379 = ct{1864};
t3380 = ct{1865};
t3381 = ct{1866};
t3384 = ct{1867};
t3385 = ct{1868};
t3388 = ct{1869};
t3390 = ct{1870};
t3391 = ct{1871};
t3392 = ct{1872};
t3393 = ct{1873};
t3397 = ct{1874};
t3398 = ct{1875};
t3399 = ct{1876};
t34 = ct{1877};
t3400 = ct{1878};
t3403 = ct{1879};
t3407 = ct{1880};
t3412 = ct{1881};
t3413 = ct{1882};
t3414 = ct{1883};
t3415 = ct{1884};
t3416 = ct{1885};
t3419 = ct{1886};
t3420 = ct{1887};
t3421 = ct{1888};
t3423 = ct{1889};
t3424 = ct{1890};
t3425 = ct{1891};
t3426 = ct{1892};
t3427 = ct{1893};
t3429 = ct{1894};
t3432 = ct{1895};
t3433 = ct{1896};
t3434 = ct{1897};
t3437 = ct{1898};
t3438 = ct{1899};
t3439 = ct{1900};
t3440 = ct{1901};
t3441 = ct{1902};
t3442 = ct{1903};
t3445 = ct{1904};
t3446 = ct{1905};
t3447 = ct{1906};
t3448 = ct{1907};
t3449 = ct{1908};
t3450 = ct{1909};
t3452 = ct{1910};
t3453 = ct{1911};
t3454 = ct{1912};
t3457 = ct{1913};
t3458 = ct{1914};
t3459 = ct{1915};
t3460 = ct{1916};
t3462 = ct{1917};
t3465 = ct{1918};
t3467 = ct{1919};
t3468 = ct{1920};
t3469 = ct{1921};
t3471 = ct{1922};
t3472 = ct{1923};
t3474 = ct{1924};
t3475 = ct{1925};
t3478 = ct{1926};
t3479 = ct{1927};
t3480 = ct{1928};
t3481 = ct{1929};
t3483 = ct{1930};
t3484 = ct{1931};
t3485 = ct{1932};
t3486 = ct{1933};
t3487 = ct{1934};
t3488 = ct{1935};
t3489 = ct{1936};
t3490 = ct{1937};
t3492 = ct{1938};
t3495 = ct{1939};
t3496 = ct{1940};
t3499 = ct{1941};
t3500 = ct{1942};
t3501 = ct{1943};
t3502 = ct{1944};
t3504 = ct{1945};
t3506 = ct{1946};
t3509 = ct{1947};
t3512 = ct{1948};
t3513 = ct{1949};
t3515 = ct{1950};
t3516 = ct{1951};
t3517 = ct{1952};
t3518 = ct{1953};
t3520 = ct{1954};
t3521 = ct{1955};
t3522 = ct{1956};
t3523 = ct{1957};
t3524 = ct{1958};
t3527 = ct{1959};
t3528 = ct{1960};
t3529 = ct{1961};
t3530 = ct{1962};
t3531 = ct{1963};
t3532 = ct{1964};
t3534 = ct{1965};
t3535 = ct{1966};
t3536 = ct{1967};
t3537 = ct{1968};
t3539 = ct{1969};
t3541 = ct{1970};
t3542 = ct{1971};
t3543 = ct{1972};
t3544 = ct{1973};
t3545 = ct{1974};
t3547 = ct{1975};
t3548 = ct{1976};
t3550 = ct{1977};
t3551 = ct{1978};
t3552 = ct{1979};
t3553 = ct{1980};
t3554 = ct{1981};
t3556 = ct{1982};
t3557 = ct{1983};
t3558 = ct{1984};
t3559 = ct{1985};
t3562 = ct{1986};
t3563 = ct{1987};
t3564 = ct{1988};
t3565 = ct{1989};
t3569 = ct{1990};
t3570 = ct{1991};
t3571 = ct{1992};
t3574 = ct{1993};
t3575 = ct{1994};
t3576 = ct{1995};
t3579 = ct{1996};
t3581 = ct{1997};
t3582 = ct{1998};
t3583 = ct{1999};
t3584 = ct{2000};
t3585 = ct{2001};
t3586 = ct{2002};
t3587 = ct{2003};
t3588 = ct{2004};
t3590 = ct{2005};
t3592 = ct{2006};
t3593 = ct{2007};
t3595 = ct{2008};
t3596 = ct{2009};
t3597 = ct{2010};
t3598 = ct{2011};
t3599 = ct{2012};
t3600 = ct{2013};
t3602 = ct{2014};
t3603 = ct{2015};
t3604 = ct{2016};
t3605 = ct{2017};
t3606 = ct{2018};
t3607 = ct{2019};
t3608 = ct{2020};
t3609 = ct{2021};
t3611 = ct{2022};
t3613 = ct{2023};
t3614 = ct{2024};
t3617 = ct{2025};
t3619 = ct{2026};
t3620 = ct{2027};
t3621 = ct{2028};
t3623 = ct{2029};
t3625 = ct{2030};
t3626 = ct{2031};
t3627 = ct{2032};
t3628 = ct{2033};
t3629 = ct{2034};
t3630 = ct{2035};
t3631 = ct{2036};
t3632 = ct{2037};
t3635 = ct{2038};
t3636 = ct{2039};
t3637 = ct{2040};
t3638 = ct{2041};
t3639 = ct{2042};
t3640 = ct{2043};
t3641 = ct{2044};
t3643 = ct{2045};
t3644 = ct{2046};
t3645 = ct{2047};
t3647 = ct{2048};
t3648 = ct{2049};
t3649 = ct{2050};
t3651 = ct{2051};
t3652 = ct{2052};
t3653 = ct{2053};
t3654 = ct{2054};
t3655 = ct{2055};
t3656 = ct{2056};
t3657 = ct{2057};
t3659 = ct{2058};
t3660 = ct{2059};
t3661 = ct{2060};
t3663 = ct{2061};
t3664 = ct{2062};
t3666 = ct{2063};
t3667 = ct{2064};
t3668 = ct{2065};
t3669 = ct{2066};
t3671 = ct{2067};
t3672 = ct{2068};
t3673 = ct{2069};
t3674 = ct{2070};
t3675 = ct{2071};
t3676 = ct{2072};
t3677 = ct{2073};
t3678 = ct{2074};
t3679 = ct{2075};
t3680 = ct{2076};
t3683 = ct{2077};
t3684 = ct{2078};
t3686 = ct{2079};
t3687 = ct{2080};
t3688 = ct{2081};
t3689 = ct{2082};
t3692 = ct{2083};
t3694 = ct{2084};
t3695 = ct{2085};
t3698 = ct{2086};
t3699 = ct{2087};
t3700 = ct{2088};
t3701 = ct{2089};
t3702 = ct{2090};
t3704 = ct{2091};
t3706 = ct{2092};
t3708 = ct{2093};
t3709 = ct{2094};
t3710 = ct{2095};
t3711 = ct{2096};
t3713 = ct{2097};
t3714 = ct{2098};
t3716 = ct{2099};
t3717 = ct{2100};
t3720 = ct{2101};
t3721 = ct{2102};
t3722 = ct{2103};
t3723 = ct{2104};
t3724 = ct{2105};
t3725 = ct{2106};
t3726 = ct{2107};
t3727 = ct{2108};
t3728 = ct{2109};
t3729 = ct{2110};
t3730 = ct{2111};
t3731 = ct{2112};
t3733 = ct{2113};
t3734 = ct{2114};
t3735 = ct{2115};
t3736 = ct{2116};
t3737 = ct{2117};
t3739 = ct{2118};
t3742 = ct{2119};
t3744 = ct{2120};
t3745 = ct{2121};
t3746 = ct{2122};
t3747 = ct{2123};
t3749 = ct{2124};
t375 = ct{2125};
t3750 = ct{2126};
t3752 = ct{2127};
t3753 = ct{2128};
t3754 = ct{2129};
t3759 = ct{2130};
t376 = ct{2131};
t3761 = ct{2132};
t3762 = ct{2133};
t3768 = ct{2134};
t3769 = ct{2135};
t377 = ct{2136};
t3770 = ct{2137};
t3771 = ct{2138};
t3772 = ct{2139};
t3773 = ct{2140};
t3775 = ct{2141};
t3776 = ct{2142};
t3777 = ct{2143};
t3778 = ct{2144};
t3779 = ct{2145};
t3780 = ct{2146};
t3781 = ct{2147};
t3783 = ct{2148};
t3784 = ct{2149};
t3785 = ct{2150};
t3786 = ct{2151};
t3787 = ct{2152};
t3789 = ct{2153};
t3790 = ct{2154};
t3791 = ct{2155};
t3792 = ct{2156};
t3793 = ct{2157};
t3794 = ct{2158};
t3795 = ct{2159};
t3796 = ct{2160};
t3799 = ct{2161};
t38 = ct{2162};
t3801 = ct{2163};
t3802 = ct{2164};
t3803 = ct{2165};
t3804 = ct{2166};
t3805 = ct{2167};
t3806 = ct{2168};
t3807 = ct{2169};
t3808 = ct{2170};
t381 = ct{2171};
t3814 = ct{2172};
t3815 = ct{2173};
t3819 = ct{2174};
t382 = ct{2175};
t3822 = ct{2176};
t3823 = ct{2177};
t3828 = ct{2178};
t383 = ct{2179};
t3832 = ct{2180};
t3836 = ct{2181};
t3838 = ct{2182};
t3842 = ct{2183};
t3843 = ct{2184};
t3844 = ct{2185};
t3845 = ct{2186};
t3846 = ct{2187};
t3847 = ct{2188};
t3851 = ct{2189};
t3854 = ct{2190};
t3855 = ct{2191};
t3858 = ct{2192};
t3859 = ct{2193};
t3862 = ct{2194};
t3866 = ct{2195};
t3871 = ct{2196};
t3873 = ct{2197};
t3877 = ct{2198};
t3880 = ct{2199};
t3882 = ct{2200};
t3883 = ct{2201};
t3889 = ct{2202};
t3898 = ct{2203};
t3899 = ct{2204};
t390 = ct{2205};
t3900 = ct{2206};
t3902 = ct{2207};
t3906 = ct{2208};
t3907 = ct{2209};
t3908 = ct{2210};
t3909 = ct{2211};
t3910 = ct{2212};
t3913 = ct{2213};
t3915 = ct{2214};
t3916 = ct{2215};
t3918 = ct{2216};
t3919 = ct{2217};
t3924 = ct{2218};
t3926 = ct{2219};
t3928 = ct{2220};
t3929 = ct{2221};
t3930 = ct{2222};
t3931 = ct{2223};
t3932 = ct{2224};
t3933 = ct{2225};
t3936 = ct{2226};
t3937 = ct{2227};
t3939 = ct{2228};
t394 = ct{2229};
t3940 = ct{2230};
t3942 = ct{2231};
t3944 = ct{2232};
t3950 = ct{2233};
t3952 = ct{2234};
t3955 = ct{2235};
t3956 = ct{2236};
t3957 = ct{2237};
t3959 = ct{2238};
t3960 = ct{2239};
t3961 = ct{2240};
t3962 = ct{2241};
t3964 = ct{2242};
t3965 = ct{2243};
t3967 = ct{2244};
t3969 = ct{2245};
t3971 = ct{2246};
t3974 = ct{2247};
t3976 = ct{2248};
t3981 = ct{2249};
t3982 = ct{2250};
t3983 = ct{2251};
t3985 = ct{2252};
t3993 = ct{2253};
t3994 = ct{2254};
t3995 = ct{2255};
t3996 = ct{2256};
t3998 = ct{2257};
t3999 = ct{2258};
t4 = ct{2259};
t4000 = ct{2260};
t4002 = ct{2261};
t4003 = ct{2262};
t4005 = ct{2263};
t4008 = ct{2264};
t401 = ct{2265};
t4012 = ct{2266};
t4014 = ct{2267};
t4023 = ct{2268};
t4024 = ct{2269};
t4028 = ct{2270};
t4029 = ct{2271};
t4033 = ct{2272};
t4035 = ct{2273};
t4036 = ct{2274};
t4038 = ct{2275};
t4042 = ct{2276};
t4045 = ct{2277};
t4046 = ct{2278};
t4047 = ct{2279};
t4048 = ct{2280};
t4049 = ct{2281};
t4051 = ct{2282};
t4052 = ct{2283};
t4053 = ct{2284};
t4054 = ct{2285};
t4055 = ct{2286};
t4056 = ct{2287};
t4058 = ct{2288};
t4059 = ct{2289};
t4060 = ct{2290};
t4061 = ct{2291};
t4064 = ct{2292};
t4067 = ct{2293};
t4068 = ct{2294};
t4069 = ct{2295};
t4070 = ct{2296};
t4071 = ct{2297};
t4072 = ct{2298};
t4073 = ct{2299};
t4074 = ct{2300};
t4075 = ct{2301};
t4076 = ct{2302};
t4078 = ct{2303};
t4079 = ct{2304};
t4081 = ct{2305};
t4086 = ct{2306};
t4087 = ct{2307};
t4089 = ct{2308};
t4090 = ct{2309};
t4092 = ct{2310};
t4093 = ct{2311};
t4094 = ct{2312};
t4095 = ct{2313};
t4097 = ct{2314};
t4098 = ct{2315};
t4099 = ct{2316};
t41 = ct{2317};
t410 = ct{2318};
t4100 = ct{2319};
t4101 = ct{2320};
t4104 = ct{2321};
t4109 = ct{2322};
t411 = ct{2323};
t4112 = ct{2324};
t4118 = ct{2325};
t4119 = ct{2326};
t412 = ct{2327};
t4121 = ct{2328};
t4122 = ct{2329};
t4123 = ct{2330};
t4124 = ct{2331};
t4125 = ct{2332};
t4126 = ct{2333};
t413 = ct{2334};
t4130 = ct{2335};
t4134 = ct{2336};
t4135 = ct{2337};
t4137 = ct{2338};
t414 = ct{2339};
t4140 = ct{2340};
t4141 = ct{2341};
t4143 = ct{2342};
t4146 = ct{2343};
t415 = ct{2344};
t4153 = ct{2345};
t4155 = ct{2346};
t4156 = ct{2347};
t4157 = ct{2348};
t4158 = ct{2349};
t4159 = ct{2350};
t4164 = ct{2351};
t4165 = ct{2352};
t4169 = ct{2353};
t4171 = ct{2354};
t4174 = ct{2355};
t4175 = ct{2356};
t4182 = ct{2357};
t4188 = ct{2358};
t4189 = ct{2359};
t4190 = ct{2360};
t4196 = ct{2361};
t4197 = ct{2362};
t4198 = ct{2363};
t420 = ct{2364};
t4203 = ct{2365};
t421 = ct{2366};
t4210 = ct{2367};
t4211 = ct{2368};
t4212 = ct{2369};
t4213 = ct{2370};
t4217 = ct{2371};
t4218 = ct{2372};
t4222 = ct{2373};
t4224 = ct{2374};
t4225 = ct{2375};
t4226 = ct{2376};
t4227 = ct{2377};
t4231 = ct{2378};
t4232 = ct{2379};
t4234 = ct{2380};
t4236 = ct{2381};
t4237 = ct{2382};
t4240 = ct{2383};
t4241 = ct{2384};
t4246 = ct{2385};
t4247 = ct{2386};
t425 = ct{2387};
t4253 = ct{2388};
t4256 = ct{2389};
t4269 = ct{2390};
t4270 = ct{2391};
t4274 = ct{2392};
t4276 = ct{2393};
t4282 = ct{2394};
t4286 = ct{2395};
t4290 = ct{2396};
t4295 = ct{2397};
t4298 = ct{2398};
t430 = ct{2399};
t4300 = ct{2400};
t4301 = ct{2401};
t4304 = ct{2402};
t4306 = ct{2403};
t431 = ct{2404};
t4312 = ct{2405};
t4316 = ct{2406};
t4323 = ct{2407};
t4324 = ct{2408};
t4325 = ct{2409};
t4326 = ct{2410};
t433 = ct{2411};
t4330 = ct{2412};
t4332 = ct{2413};
t4339 = ct{2414};
t4342 = ct{2415};
t4348 = ct{2416};
t4349 = ct{2417};
t4354 = ct{2418};
t4355 = ct{2419};
t4356 = ct{2420};
t4358 = ct{2421};
t436 = ct{2422};
t4364 = ct{2423};
t4367 = ct{2424};
t4368 = ct{2425};
t4371 = ct{2426};
t4393 = ct{2427};
t4395 = ct{2428};
t44 = ct{2429};
t4406 = ct{2430};
t4418 = ct{2431};
t4420 = ct{2432};
t4421 = ct{2433};
t4424 = ct{2434};
t4432 = ct{2435};
t445 = ct{2436};
t4453 = ct{2437};
t4454 = ct{2438};
t4457 = ct{2439};
t4458 = ct{2440};
t4464 = ct{2441};
t4475 = ct{2442};
t4477 = ct{2443};
t4479 = ct{2444};
t4481 = ct{2445};
t4487 = ct{2446};
t4490 = ct{2447};
t4492 = ct{2448};
t4495 = ct{2449};
t4496 = ct{2450};
t4497 = ct{2451};
t450 = ct{2452};
t4506 = ct{2453};
t451 = ct{2454};
t4512 = ct{2455};
t4525 = ct{2456};
t4538 = ct{2457};
t4545 = ct{2458};
t4549 = ct{2459};
t4551 = ct{2460};
t4581 = ct{2461};
t459 = ct{2462};
t4597 = ct{2463};
t4598 = ct{2464};
t46 = ct{2465};
t4602 = ct{2466};
t4603 = ct{2467};
t4628 = ct{2468};
t4646 = ct{2469};
t4649 = ct{2470};
t465 = ct{2471};
t4659 = ct{2472};
t4665 = ct{2473};
t4695 = ct{2474};
t4711 = ct{2475};
t4732 = ct{2476};
t4739 = ct{2477};
t4740 = ct{2478};
t4752 = ct{2479};
t4789 = ct{2480};
t4796 = ct{2481};
t48 = ct{2482};
t482 = ct{2483};
t483 = ct{2484};
t484 = ct{2485};
t485 = ct{2486};
t487 = ct{2487};
t4873 = ct{2488};
t488 = ct{2489};
t49 = ct{2490};
t4909 = ct{2491};
t491 = ct{2492};
t4925 = ct{2493};
t4931 = ct{2494};
t4932 = ct{2495};
t4936 = ct{2496};
t4944 = ct{2497};
t4953 = ct{2498};
t4954 = ct{2499};
t496 = ct{2500};
t4976 = ct{2501};
t4995 = ct{2502};
t5 = ct{2503};
t50 = ct{2504};
t501 = ct{2505};
t502 = ct{2506};
t5021 = ct{2507};
t5032 = ct{2508};
t504 = ct{2509};
t5053 = ct{2510};
t5054 = ct{2511};
t5058 = ct{2512};
t5059 = ct{2513};
t5066 = ct{2514};
t51 = ct{2515};
t514 = ct{2516};
t519 = ct{2517};
t5200 = ct{2518};
t5208 = ct{2519};
t5227 = ct{2520};
t523 = ct{2521};
t524 = ct{2522};
t5265 = ct{2523};
t527 = ct{2524};
t5275 = ct{2525};
t530 = ct{2526};
t5317 = ct{2527};
t534 = ct{2528};
t537 = ct{2529};
t539 = ct{2530};
t5399 = ct{2531};
t54 = ct{2532};
t541 = ct{2533};
t542 = ct{2534};
t5420 = ct{2535};
t5424 = ct{2536};
t5431 = ct{2537};
t5438 = ct{2538};
t544 = ct{2539};
t546 = ct{2540};
t55 = ct{2541};
t550 = ct{2542};
t553 = ct{2543};
t5539 = ct{2544};
t557 = ct{2545};
t5572 = ct{2546};
t5576 = ct{2547};
t558 = ct{2548};
t56 = ct{2549};
t5674 = ct{2550};
t57 = ct{2551};
t5706 = ct{2552};
t573 = ct{2553};
t574 = ct{2554};
t575 = ct{2555};
t587 = ct{2556};
t59 = ct{2557};
t595 = ct{2558};
t603 = ct{2559};
t61 = ct{2560};
t614 = ct{2561};
t623 = ct{2562};
t624 = ct{2563};
t627 = ct{2564};
t628 = ct{2565};
t629 = ct{2566};
t632 = ct{2567};
t634 = ct{2568};
t641 = ct{2569};
t644 = ct{2570};
t65 = ct{2571};
t650 = ct{2572};
t651 = ct{2573};
t655 = ct{2574};
t657 = ct{2575};
t664 = ct{2576};
t665 = ct{2577};
t666 = ct{2578};
t667 = ct{2579};
t668 = ct{2580};
t669 = ct{2581};
t674 = ct{2582};
t675 = ct{2583};
t68 = ct{2584};
t693 = ct{2585};
t699 = ct{2586};
t7 = ct{2587};
t71 = ct{2588};
t720 = ct{2589};
t721 = ct{2590};
t724 = ct{2591};
t73 = ct{2592};
t731 = ct{2593};
t732 = ct{2594};
t735 = ct{2595};
t736 = ct{2596};
t741 = ct{2597};
t744 = ct{2598};
t746 = ct{2599};
t749 = ct{2600};
t752 = ct{2601};
t753 = ct{2602};
t754 = ct{2603};
t755 = ct{2604};
t756 = ct{2605};
t757 = ct{2606};
t759 = ct{2607};
t760 = ct{2608};
t761 = ct{2609};
t762 = ct{2610};
t764 = ct{2611};
t765 = ct{2612};
t769 = ct{2613};
t772 = ct{2614};
t774 = ct{2615};
t776 = ct{2616};
t778 = ct{2617};
t779 = ct{2618};
t792 = ct{2619};
t795 = ct{2620};
t797 = ct{2621};
t799 = ct{2622};
t8 = ct{2623};
t802 = ct{2624};
t803 = ct{2625};
t806 = ct{2626};
t811 = ct{2627};
t817 = ct{2628};
t818 = ct{2629};
t820 = ct{2630};
t821 = ct{2631};
t823 = ct{2632};
t824 = ct{2633};
t828 = ct{2634};
t831 = ct{2635};
t834 = ct{2636};
t837 = ct{2637};
t838 = ct{2638};
t839 = ct{2639};
t841 = ct{2640};
t842 = ct{2641};
t843 = ct{2642};
t844 = ct{2643};
t845 = ct{2644};
t846 = ct{2645};
t847 = ct{2646};
t848 = ct{2647};
t850 = ct{2648};
t851 = ct{2649};
t852 = ct{2650};
t853 = ct{2651};
t854 = ct{2652};
t855 = ct{2653};
t864 = ct{2654};
t865 = ct{2655};
t867 = ct{2656};
t868 = ct{2657};
t870 = ct{2658};
t871 = ct{2659};
t872 = ct{2660};
t874 = ct{2661};
t875 = ct{2662};
t876 = ct{2663};
t877 = ct{2664};
t885 = ct{2665};
t886 = ct{2666};
t888 = ct{2667};
t889 = ct{2668};
t890 = ct{2669};
t891 = ct{2670};
t892 = ct{2671};
t893 = ct{2672};
t896 = ct{2673};
t897 = ct{2674};
t898 = ct{2675};
t9 = ct{2676};
t901 = ct{2677};
t902 = ct{2678};
t903 = ct{2679};
t904 = ct{2680};
t906 = ct{2681};
t907 = ct{2682};
t908 = ct{2683};
t909 = ct{2684};
t912 = ct{2685};
t914 = ct{2686};
t915 = ct{2687};
t916 = ct{2688};
t918 = ct{2689};
t923 = ct{2690};
t924 = ct{2691};
t925 = ct{2692};
t926 = ct{2693};
t927 = ct{2694};
t928 = ct{2695};
t934 = ct{2696};
t947 = ct{2697};
t949 = ct{2698};
t950 = ct{2699};
t951 = ct{2700};
t952 = ct{2701};
t953 = ct{2702};
t954 = ct{2703};
t955 = ct{2704};
t957 = ct{2705};
t964 = ct{2706};
t965 = ct{2707};
t970 = ct{2708};
t972 = ct{2709};
t977 = ct{2710};
t979 = ct{2711};
t980 = ct{2712};
t983 = ct{2713};
t985 = ct{2714};
t987 = ct{2715};
t991 = ct{2716};
t992 = ct{2717};
t993 = ct{2718};
t994 = ct{2719};
t995 = ct{2720};
t996 = ct{2721};
t3809 = t2641.*9.52624335e-4;
t3811 = t1510.*t2116;
t3812 = t2641.*3.372816795e-3;
t3816 = t2826.*3.36554e-3;
t3817 = t2827.*3.36554e-3;
t3821 = t2831.*3.36554e-3;
t3826 = Mt.*t5.*t9.*t3679;
t3833 = -t3822;
t3837 = t2899.*3.36554e-3;
t3841 = Mt.*t1381.*t2319;
t3849 = Mt.*t4.*t5.*t3780;
t3850 = Mt.*t9.*t10.*t3780;
t3863 = t2826.*9.52624335e-4;
t3864 = t2827.*9.52624335e-4;
t3867 = t2831.*9.52624335e-4;
t3868 = t2831.*1.90524867e-3;
t3869 = t2826.*3.372816795e-3;
t3870 = t2827.*3.372816795e-3;
t3874 = t2831.*3.372816795e-3;
t3875 = t2831.*6.74563359e-3;
t3878 = dpsi1.*t3836;
t3879 = t1510.*t2327;
t3890 = -t3877;
t3894 = Mt.*t5.*t33.*t3780;
t3896 = Mt.*t5.*t38.*t3780;
t3897 = t2899.*9.52624335e-4;
t3903 = t2899.*3.372816795e-3;
t3922 = -t3113.*(t214-t541);
t3923 = -B_cg_H.*Mb.*t3082.*(t197-t537);
t3927 = Mb.*t4.*t10.*t3836;
t3935 = -t3924;
t3938 = t918+t1527+t1604;
t3941 = Mt.*t382.*t3679;
t3948 = t1047.*t3113;
t3949 = Mb.*t5.*t30.*t3836;
t3953 = B_cg_H.*Mb.*t3082.*(t197-t537);
t3954 = Mb.*t5.*t34.*t3836;
t3966 = t3195.*3.36554e-3;
t3970 = Mt.*t420.*t3679;
t3980 = B_cg_H.*Mb.*t1510.*t2563;
t3990 = Mb.*t1558.*t2527;
t3991 = Mt.*t381.*t3780;
t3992 = Mt.*t382.*t3780;
t4011 = -t3999;
t4013 = -t4002;
t4020 = Mt.*t420.*t3780;
t4021 = Mt.*t421.*t3780;
t4025 = Mt.*t1727.*t2319;
t4026 = B_cg_H.*Mb.*t1510.*t2638;
t4027 = t1178.*t3113;
t4031 = t3195.*9.52624335e-4;
t4034 = t3195.*3.372816795e-3;
t4050 = Mb.*t381.*t3836;
t4063 = t644+t720+t934+t1026+t1107;
t4066 = Mb.*t421.*t3836;
t4080 = t674+t731+t927+t1099+t1113;
t4083 = -t4075;
t4084 = -t4076;
t4085 = B_cg_H.*Mb.*t11.*t459.*t3836;
t4096 = t1430.*t3113;
t4102 = B_cg_H.*Mb.*t1512.*t3082;
t4105 = t1510.*t3143;
t4108 = B_cg_H.*Mb.*t675.*t3836;
t4111 = t1512.*t3113;
t4115 = t483+t792+t909+t1169+t1288;
t4128 = -t1510.*(-t488+t603+dpsi1.*(t105-t465)+dth2.*(t103-t544));
t4132 = t482+t623+t624+t752+t908+t1286;
t4133 = Mb.*t1558.*t3138;
t4144 = -t4134;
t4145 = -t4135;
t4150 = Mt.*t5.*t9.*t4100;
t4151 = t1510.*(-t488+t603+dpsi1.*(t105-t465)+dth2.*(t103-t544)).*(-1.0./2.0);
t4160 = Mt.*t2319.*t2325;
t4173 = t2309+t2449;
t4177 = -t4157;
t4187 = B_cg_H.*Mb.*t977.*t3836;
t4191 = -t4174;
t4193 = -t4175;
t4201 = B_cg_H.*Mb.*t1037.*t3836;
t4204 = -B_cg_H.*Mb.*t3836.*(t195-t634);
t4216 = -t4198;
t4220 = B_cg_H.*Mb.*t3836.*(t195-t634);
t4221 = Mt.*t382.*t4100;
t4223 = t3113.*(t214-t541).*(-3.36554e-3);
t4228 = Mt.*t2319.*t2763;
t4230 = Mt.*t420.*t4100;
t4239 = B_cg_H.*Mb.*t1179.*t3836;
t4242 = t1355+t1796+t1833;
t4248 = -t4225;
t4249 = -t4226;
t4254 = t947+t1988+t2028;
t4255 = t1061+t1933+t1935;
t4261 = -t4246;
t4262 = -Mt.*t2914.*(t433-t828+T_cg_H.*(t197-t537));
t4263 = Mt.*t2319.*t2915;
t4264 = t699+t779+t1226+t1229+t1297;
t4268 = Mt.*t1528.*t3780;
t4272 = t903.*t4079;
t4273 = Mt.*t2319.*(-t120+t425+t519-t651+t765);
t4292 = Mb.*t1558.*t3836;
t4293 = t1017+t2126+t2167;
t4299 = t811+t864+t1231+t1295+t1340;
t4305 = Mt.*t1734.*t3780;
t4307 = Mb.*t2563.*t3082;
t4308 = -t4300;
t4311 = t1323+t1992+t2014;
t4320 = Mb.*t1660.*t3836;
t4328 = t1510.*(-t488+t603+dpsi1.*(t105-t465)+dth2.*(t103-t544)).*(-3.36554e-3);
t4333 = t1510.*(-t488+t603+dpsi1.*(t105-t465)+dth2.*(t103-t544)).*3.36554e-3;
t4334 = -t4325;
t4338 = t1510.*(-t488+t603+dpsi1.*(t105-t465)+dth2.*(t103-t544)).*(-3.367829185e-3);
t4344 = t46+t123+t484+t627+t735+t3679;
t4345 = t1510.*(-t488+t603+dpsi1.*(t105-t465)+dth2.*(t103-t544)).*3.367829185e-3;
t4346 = t28+t57+t160+t632+t951+t1519+t2063;
t4351 = t1510.*(-t488+t603+dpsi1.*(t105-t465)+dth2.*(t103-t544)).*(-8.56645e-6);
t4360 = -Mt.*t3679.*(t433-t828+T_cg_H.*(t197-t537));
t4361 = Mt.*t2174.*t3780;
t4365 = Mt.*t3679.*(t433-t828+T_cg_H.*(t197-t537));
t4372 = -Mt.*t3780.*(t451-t831+T_cg_H.*(t214-t541));
t4375 = Mt.*t2319.*t3780;
t4381 = t1325+t2314+t2364;
t4382 = t1324+t2239+t2443;
t4390 = -t4270.*(t105-t465);
t4399 = t4270.*(t105-t465);
t4402 = -t4395;
t4408 = t1451+t2378+t2446;
t4414 = Mt.*t2730.*t3780;
t4416 = t1408+t2344+t2596;
t4422 = t970+t980+t1293+t1571+t1580;
t4423 = t375+t893+t897+t985+t1625+t1666;
t4425 = Mt.*t2319.*t3937;
t4427 = Mb.*t2638.*t3836;
t4428 = Mt.*t2325.*t3940;
t4430 = t1439+t2432+t2524;
t4436 = t4300.*3.36554e-3;
t4437 = t1041+t1046+t1225+t1570+t1581;
t4438 = -t4424;
t4440 = Mt.*t2914.*t3780;
t4441 = Mt.*t2319.*t3971;
t4449 = Mt.*t3780.*(-t130+t436+t523-t657+t769);
t4461 = t1653+t2631+t2643;
t4467 = Mt.*t2914.*t3937;
t4468 = t401+t746+t823+t1045+t1842+t1984;
t4469 = -Mt.*t4100.*(t433-t828+T_cg_H.*(t197-t537));
t4472 = -t4464;
t4476 = t1515+t2770+t2827;
t4478 = -t1505.*(-t724-t778+t1230+t1291+dphi2.*(t534-t546));
t4486 = Mt.*t4100.*(t433-t828+T_cg_H.*(t197-t537));
t4488 = Mt.*t2325.*t4112;
t4494 = t1437+t2831+t2900;
t4514 = t4393.*3.36554e-3;
t4516 = t4395.*3.36554e-3;
t4527 = t993+t1542+t1552+t1584+t1592;
t4529 = -t4525;
t4552 = -t4545;
t4558 = Mt.*t3679.*t3937;
t4561 = Mt.*t3780.*t3940;
t4569 = t514+t1114+t1127+t1128+t1877+t1920;
t4571 = Mt.*t3780.*t3969;
t4575 = t1812+t1819+t1953+t2030;
t4583 = t1505.*(-t724-t778+t1230+t1291+dphi2.*(t534-t546)).*(-3.36554e-3);
t4611 = Mt.*t3780.*t4100;
t4612 = t2388+t3020+t3044;
t4616 = Mt.*t3780.*t4112;
t4632 = t1057+t1733+t1742+t1834+t1856;
t4641 = dth2.*t4628;
t4654 = t1974+t3364+t3369;
t4655 = Mt.*t3937.*t4100;
t4686 = t821+t1055+t1367+t1445+t1923+t2121;
t4707 = ITail.*t3961.*t4227;
t4709 = ITail.*t4071.*t4164;
t4713 = -ITail.*t4072.*(-t1262+t1701+t9.*t868.*(t105-t465));
t4719 = t839+t1056+t1704+t1771+t1926+t1957;
t4722 = t1154+t1461+t1539+t1583+t1732+t1873;
t4723 = ITail.*t3961.*t4286;
t4724 = ITail.*t4071.*t4237;
t4731 = -ITail.*t4072.*(-t947+t1240.*(t105-t465)+t903.*(t534-t546));
t4733 = ITail.*t4072.*(-t947+t1240.*(t105-t465)+t903.*(t534-t546));
t4735 = t1383+t1409+t1537+t1547+t1803+t1835;
t4736 = t2612+t3590+t3781;
t4745 = dth2.*t4739;
t4746 = dth2.*t4740;
t4762 = t845+t1125+t1282+t1715+t2396+t2795;
t4772 = -ITail.*t4237.*(-t1355+t1789+(t9.*t868.*(t105-t465))./2.0);
t4774 = -ITail.*t4227.*(-t947+t1240.*(t105-t465)+t903.*(t534-t546));
t4776 = -ITail.*t4286.*(-t1262+t1701+t9.*t868.*(t105-t465));
t4784 = ITail.*t4227.*(-t947+t1240.*(t105-t465)+t903.*(t534-t546));
t4802 = -ITail.*t4071.*(t1260-t2364+t1430.*(t105-t465));
t4809 = ITail.*t4071.*(t1260-t2364+t1430.*(t105-t465));
t4821 = t1139+t1177+t1987+t1994+t2099+t2100;
t4823 = t1320+t1450+t1811+t1866+t2105+t2114;
t4848 = ITail.*(t1260-t2364+t1430.*(t105-t465)).*(-t1355+t1789+(t9.*t868.*(t105-t465))./2.0);
t4849 = t1131+t1522+t1816+t1825+t2373+t2442;
t4866 = t889+t1419+t1482+t1769+t2851+t3036;
t4878 = dphi2.*t4873;
t4885 = t923+t1360+t1561+t1827+t2791+t3095;
t4889 = -dth2.*(t886-t1360+t1759-t2791+Mt.*t421.*(t431+t909+T_cg_H.*(t195-t634))+B_cg_H.*Mb.*t421.*(t195-t634));
t4895 = ITail.*(t1260-t2364+t1430.*(t105-t465)).*(-t1017+(t1240.*(t105-t465))./2.0+(t903.*(t534-t546))./2.0);
t4913 = -ITail.*t4490.*(-t1262+t1701+t9.*t868.*(t105-t465));
t4922 = t1442+t1520+t2187+t2265+t2267+t2272;
t4923 = t1616+t1654+t1913+t1919+t2365+t2377;
t4933 = -ITail.*t4490.*(-t947+t1240.*(t105-t465)+t903.*(t534-t546));
t4938 = t3961.*t4602;
t4942 = t4164.*t4551;
t4945 = ITail.*t4071.*t4581;
t4946 = -t4549.*(-t1262+t1701+t9.*t868.*(t105-t465));
t4964 = ITail.*t3961.*t4646;
t4965 = t2058+t2704+t2718+t2739+t2747;
t4966 = t3961.*t4649;
t4967 = t4237.*t4551;
t4970 = -t4549.*(-t947+t1240.*(t105-t465)+t903.*(t534-t546));
t4975 = t4549.*(-t947+t1240.*(t105-t465)+t903.*(t534-t546));
t4986 = t1010+t1559+t1577+t2328+t3274+t3295;
t4987 = t1012+t1560+t1576+t2331+t3275+t3294;
t4988 = -ITail.*t4071.*(t1751+t2308+t964.*(t105-t465)+t1430.*(t103-t544));
t4993 = ITail.*t4071.*(t1751+t2308+t964.*(t105-t465)+t1430.*(t103-t544));
t5036 = -t4237.*(-t2388+t3008+t9.*t868.*(t105-t465).*9.53094055e-4);
t5037 = -t4602.*(-t947+t1240.*(t105-t465)+t903.*(t534-t546));
t5042 = -t4649.*(-t1262+t1701+t9.*t868.*(t105-t465));
t5046 = t4602.*(-t947+t1240.*(t105-t465)+t903.*(t534-t546));
t5051 = ITail.*t4071.*t4695;
t5067 = -t4551.*(t1260-t2364+t1430.*(t105-t465));
t5072 = -ITail.*t4071.*(t1260-t1328-t1427-t1441+t1706+t9.*t870.*(t105-t465));
t5078 = ITail.*(-t1355+t1789+(t9.*t868.*(t105-t465))./2.0).*(t1751+t2308+t964.*(t105-t465)+t1430.*(t103-t544));
t5080 = t4551.*(t1260-t2364+t1430.*(t105-t465));
t5083 = -ITail.*t4646.*(-t947+t1240.*(t105-t465)+t903.*(t534-t546));
t5086 = t2098+t2951+t2952+t3045+t3081;
t5092 = ITail.*t4646.*(-t947+t1240.*(t105-t465)+t903.*(t534-t546));
t5103 = -ITail.*t4071.*(t753+t991-t1771-t1957+t1181.*(t105-t465)+t11.*t381.*(t534-t546));
t5109 = ITail.*(-t1017+(t1240.*(t105-t465))./2.0+(t903.*(t534-t546))./2.0).*(t1751+t2308+t964.*(t105-t465)+t1430.*(t103-t544));
t5153 = (t1260-t2364+t1430.*(t105-t465)).*(-t2388+t3008+t9.*t868.*(t105-t465).*9.53094055e-4);
t5179 = -ITail.*t4695.*(-t1017+(t1240.*(t105-t465))./2.0+(t903.*(t534-t546))./2.0);
t5198 = ITail.*(-t1355+t1789+(t9.*t868.*(t105-t465))./2.0).*(t753+t991-t1771-t1957+t1181.*(t105-t465)+t11.*t381.*(t534-t546));
t5202 = (t1260-t2364+t1430.*(t105-t465)).*(-t1974+t1240.*(t105-t465).*9.53094055e-4+t903.*(t534-t546).*9.53094055e-4);
t5206 = -t5200;
t5300 = t4551.*t4581;
t5331 = t2135+t2520+t2699+t2738+t2950+t3105;
t5351 = t2423+t2466+t2695+t2711+t3023+t3046;
t5358 = -t4551.*(t1751+t2308+t964.*(t105-t465)+t1430.*(t103-t544));
t5363 = t4551.*(t1751+t2308+t964.*(t105-t465)+t1430.*(t103-t544));
t5427 = t4551.*t4695;
t5433 = dphi1.*t5424;
t5448 = -t4551.*(t1260-t1328-t1427-t1441+t1706+t9.*t870.*(t105-t465));
t5453 = (-t2388+t3008+t9.*t868.*(t105-t465).*9.53094055e-4).*(t1751+t2308+t964.*(t105-t465)+t1430.*(t103-t544));
t5476 = -t4551.*(t753+t991-t1771-t1957+t1181.*(t105-t465)+t11.*t381.*(t534-t546));
t5488 = (-t1974+t1240.*(t105-t465).*9.53094055e-4+t903.*(t534-t546).*9.53094055e-4).*(t1751+t2308+t964.*(t105-t465)+t1430.*(t103-t544));
t5498 = -t4936.*(-t1262+t1701+t9.*t868.*(t105-t465));
t5530 = -t4936.*(-t947+t1240.*(t105-t465)+t903.*(t534-t546));
t5547 = -t4695.*(-t1974+t1240.*(t105-t465).*9.53094055e-4+t903.*(t534-t546).*9.53094055e-4);
t5565 = (-t2388+t3008+t9.*t868.*(t105-t465).*9.53094055e-4).*(t753+t991-t1771-t1957+t1181.*(t105-t465)+t11.*t381.*(t534-t546));
t5582 = -t5572;
t5598 = -t3961.*(t2449.*3.36554e-3+t3490-t3632+t1510.*(t105-t465).*3.372786875e-3);
t5690 = (-t1262+t1701+t9.*t868.*(t105-t465)).*(t2449.*3.36554e-3+t3490-t3632+t1510.*(t105-t465).*3.372786875e-3);
t5705 = t3961.*t5208;
t5716 = (-t947+t1240.*(t105-t465)+t903.*(t534-t546)).*(t2449.*3.36554e-3+t3490-t3632+t1510.*(t105-t465).*3.372786875e-3);
t5788 = t3961.*(t2135-t2468+t2699+t2738+t2950+t3105);
t5791 = -t5208.*(-t947+t1240.*(t105-t465)+t903.*(t534-t546));
t5800 = t5208.*(-t947+t1240.*(t105-t465)+t903.*(t534-t546));
t5869 = -(-t947+t1240.*(t105-t465)+t903.*(t534-t546)).*(t2135-t2468+t2699+t2738+t2950+t3105);
t6554 = t762+t1003+t1188+t1191+t1416+t1599+t1605+t2217+t2221+t2229+t2776+t3092+t3245+t3484+t3565+t3699+t4093+t4130;
t6556 = t854+t1006+t1152+t1257+t1457+t1562+t1638+t2149+t2223+t2292+t2681+t3106+t3216+t3520+t3527+t3702+t4094+t4122;
t6589 = t953+t1011+t1158+t1172+t1199+t1232+t2060+t2228+t2862+t2869+t2881+t2885+t3574+t3706+t4045+t4049+t4055+t4060;
t6599 = -dth1.*(t952-t953-t1158+t1159-t1172+t1173-t2060+t2148+t2799+t2816-t2869-t2885-t3574+t3644+t4028+t4036-t4049-t4060);
t6627 = t996+t1005+t1272+t1308+t1493+t1532+t2136+t2222+t2923+t2947+t3229+t3246+t3663+t3701+t4067+t4069+t4118+t4125;
t6629 = -dth1.*(t1004+t1008-t1206-t1247-t1459+t1492+t2142+t2225-t2849-t2878-t3175+t3228+t3628+t3704-t4052-t4058-t4101+t4124);
t1611 = B_cg_H.*t1574;
t1752 = -t1697;
t1782 = Mb.*t4.*t5.*t1622;
t1840 = -t1780;
t1853 = t1763./2.0;
t1869 = -t1848;
t1997 = -t1932;
t2003 = -t1934;
t2013 = -t1947;
t2038 = t1932./2.0;
t2040 = t1934./2.0;
t2107 = -t2012;
t2128 = t1991./2.0;
t2138 = t2001./2.0;
t2139 = t2002./2.0;
t2162 = t2019./2.0;
t2173 = -t2133;
t2195 = -t2164;
t2198 = -t2166;
t2234 = t2101./2.0;
t2243 = t2111./2.0;
t2244 = t2112./2.0;
t2250 = -t2204;
t2279 = -t2241;
t2282 = -t2197;
t2332 = -t2300;
t2391 = -t2329;
t2416 = t2313./2.0;
t2450 = -t2368;
t2451 = -t2413;
t2501 = t2368./2.0;
t2554 = -t2444;
t2558 = -t2452;
t2601 = t2444./2.0;
t2609 = t2452./2.0;
t2639 = -t2578;
t2651 = -t2593;
t2652 = -t2594;
t2676 = -t2574;
t2734 = Mb.*t15.*t2537;
t2741 = -t2642;
t2767 = -t2674;
t2780 = t2642./2.0;
t2794 = -t2728;
t2805 = -t2737;
t2905 = -t2829;
t2930 = t1763.*3.36554e-3;
t2939 = t2829./2.0;
t2965 = -t2925;
t2970 = Mb.*t15.*t2829;
t2971 = -t2933;
t3000 = t2904./2.0;
t3086 = t1763.*3.367829185e-3;
t3103 = -t3071;
t3104 = -t3073;
t3121 = t1763.*8.56645e-6;
t3155 = t1932.*3.36554e-3;
t3161 = t1934.*3.36554e-3;
t3168 = -t3101;
t3183 = -t3150;
t3219 = t1991.*3.36554e-3;
t3227 = t3192.*2.0;
t3231 = t2001.*3.36554e-3;
t3232 = t2002.*3.36554e-3;
t3234 = t3123./2.0;
t3251 = t2019.*3.36554e-3;
t3254 = -t3211;
t3258 = -t3225;
t3262 = dphi1.*t3206;
t3267 = -t3253;
t3292 = t1934.*3.372786875e-3;
t3293 = t1934.*9.53094055e-4;
t3299 = t1932.*3.367829185e-3;
t3302 = t1934.*3.367829185e-3;
t3308 = t2101.*3.36554e-3;
t3313 = t2111.*3.36554e-3;
t3314 = t2112.*3.36554e-3;
t3316 = Mb.*t4.*t5.*t3139;
t3324 = -t3255;
t3327 = -t3283;
t3342 = -t3311;
t3343 = -t3312;
t3347 = t1932.*8.56645e-6;
t3349 = t2019.*3.372786875e-3;
t3352 = t1934.*8.56645e-6;
t3355 = t2019.*9.53094055e-4;
t3377 = t2019.*3.367829185e-3;
t3382 = t1991.*3.367829185e-3;
t3386 = t2001.*3.367829185e-3;
t3387 = t2002.*3.367829185e-3;
t3396 = Mb.*t4.*t5.*t3206;
t3401 = -t3346;
t3404 = Mb.*t9.*t10.*t3206;
t3405 = -t3350;
t3406 = -t3358;
t3408 = -t3363;
t3409 = -t3371;
t3410 = -t3374;
t3430 = t2001.*8.56645e-6;
t3431 = t2002.*8.56645e-6;
t3443 = t2111.*3.367829185e-3;
t3444 = t2112.*3.367829185e-3;
t3455 = t2019.*8.56645e-6;
t3456 = t2101.*9.52624335e-4;
t3463 = t2101.*3.372816795e-3;
t3464 = t1991.*8.56645e-6;
t3466 = -t3423;
t3470 = -t3424;
t3476 = -t3432;
t3477 = -t3433;
t3491 = Mb.*t5.*t33.*t3206;
t3494 = t2313.*3.36554e-3;
t3497 = Mb.*t5.*t38.*t3206;
t3508 = -t3489;
t3510 = t2111.*8.56645e-6;
t3511 = t2112.*8.56645e-6;
t3526 = -t3481;
t3533 = -t3506;
t3538 = t2368.*3.36554e-3;
t3578 = t2313.*3.367829185e-3;
t3591 = t2444.*3.36554e-3;
t3594 = t2452.*3.36554e-3;
t3601 = -t3563;
t3610 = -t3582;
t3615 = -t3585;
t3616 = -t3586;
t3618 = Mb.*t381.*t3139;
t3622 = -t3592;
t3624 = -t3597;
t3634 = t2368.*9.53094055e-4;
t3646 = t2368.*3.367829185e-3;
t3658 = t2313.*8.56645e-6;
t3665 = t2368.*3.372786875e-3;
t3681 = Mb.*t381.*t3206;
t3682 = Mb.*t382.*t3206;
t3685 = Mb.*t421.*t3139;
t3691 = t2452.*9.52624335e-4;
t3693 = t2444.*3.372816795e-3;
t3697 = t2452.*3.372816795e-3;
t3712 = t2642.*3.36554e-3;
t3719 = t2368.*8.56645e-6;
t3732 = t2444.*9.52624335e-4;
t3741 = -t3694;
t3751 = -t3714;
t3756 = Mb.*t420.*t3206;
t3757 = Mb.*t421.*t3206;
t3760 = -t3720;
t3763 = -t3727;
t3764 = -t3728;
t3765 = -t3731;
t3767 = -t3734;
t3774 = t450+t749+t912+t1569;
t3810 = t2642.*9.52624335e-4;
t3813 = t2642.*3.372816795e-3;
t3818 = t2829.*3.36554e-3;
t3820 = -t3801;
t3829 = -t3816;
t3831 = -t3821;
t3834 = B_cg_H.*Mb.*t11.*t542.*t3206;
t3840 = t2904.*3.36554e-3;
t3848 = t41+t483+t1394+t1622;
t3856 = B_cg_H.*Mb.*t721.*t3206;
t3857 = Mt.*t4.*t5.*t3770;
t3865 = t2829.*9.52624335e-4;
t3872 = t2829.*3.372816795e-3;
t3884 = -t3863;
t3886 = -t3869;
t3887 = -t3875;
t3888 = -t3874;
t3901 = t2904.*9.52624335e-4;
t3911 = t2904.*3.372816795e-3;
t3914 = -t3878;
t3921 = -t3894;
t3934 = t3123.*3.36554e-3;
t3946 = t3192.*6.73108e-3;
t3947 = B_cg_H.*Mb.*t964.*t3139;
t3951 = B_cg_H.*Mb.*t925.*t3206;
t3958 = -t3927;
t3975 = B_cg_H.*Mb.*t964.*t3206;
t3978 = -t3948;
t3979 = -t3949;
t3984 = -t3954;
t3986 = -B_cg_H.*Mb.*t3206.*(t214-t541);
t3987 = Mt.*t381.*t3770;
t3997 = t3123.*9.52624335e-4;
t4001 = t3123.*3.372816795e-3;
t4007 = -t3980;
t4009 = B_cg_H.*Mb.*t1047.*t3206;
t4010 = B_cg_H.*Mb.*t3206.*(t214-t541);
t4015 = Mt.*t421.*t3770;
t4019 = Mb.*t1622.*t2527;
t4022 = -t3992;
t4030 = t3192.*1.90524867e-3;
t4032 = t3192.*6.74563359e-3;
t4040 = -t4020;
t4041 = -t4025;
t4043 = -t4027;
t4065 = B_cg_H.*Mb.*t1178.*t3206;
t4077 = t1049+t1626+t1662;
t4116 = Mb.*t1487.*t3206;
t4117 = B_cg_H.*Mb.*t1510.*t3139;
t4120 = -t4102;
t4129 = -t4108;
t4131 = -t4111;
t4138 = t4111./2.0;
t4139 = B_cg_H.*Mb.*t1510.*t3206;
t4147 = dphi1.*t4132;
t4152 = t3811.*3.36554e-3;
t4162 = t2374+t2375;
t4166 = Mt.*t4.*t5.*t4115;
t4168 = -t4150;
t4176 = Mt.*t4.*t5.*t4132;
t4178 = Mt.*t9.*t10.*t4132;
t4179 = -t4160;
t4184 = Mb.*t1676.*t3206;
t4192 = Mt.*t5.*t33.*t4132;
t4194 = Mt.*t5.*t38.*t4132;
t4199 = t3879.*3.36554e-3;
t4206 = -t4187;
t4214 = t2414+t2556;
t4215 = t2508+t2509;
t4229 = Mt.*t381.*t4115;
t4233 = t3948.*3.36554e-3;
t4244 = Mt.*t381.*t4132;
t4245 = Mt.*t382.*t4132;
t4250 = -t4228;
t4252 = Mt.*t421.*t4115;
t4258 = Mt.*t420.*t4132;
t4259 = Mt.*t421.*t4132;
t4267 = t4027.*3.36554e-3;
t4275 = -t4080.*(t105-t465);
t4277 = t1063+t1934+t2092;
t4278 = -t4268;
t4280 = -t4273;
t4281 = t4080.*(t105-t465);
